simulink model "battery_cell_balancing_comparison"  (R2024b)
(part 3 of 4)

  EOL TWAICE Cell Model Pair 9 : batteryecm_lib/Battery (Table-Based)  Commented=on  SOC_vec=eol_soc  T_dependence=simscape.enum.tablebattery.temperature_dependence.yes  prm_dir=simscape.enum.tablebattery.prm_dir.noCurrentDirectionality  T_vec=temp_range degC  V0_mat=eol_ocv V  V0_vec=[3.5057, 3.566, 3.6337, 3.7127, 3.9259, 4.0777, 4.1928] V  V_range=[2.8,4.15] V  R0_mat=eol_ohmic_res mOhm  R0_vec=[.0085, .0085, .0087, .0082, .0083, .0085, .0085] Ohm  R0_dis_mat=[.0117, .0085, .009; .011, .0085, .009; .0114, .0087, .0092; .0107, .0082, .0088; .0107, .0083, .0091; .0113, .0085, .0089; .0116, .0085, .0089] Ohm  R0_dis_vec=[.0085, .0085, .0087, .0082, .0083, .0085, .0085] Ohm  R0_ch_mat=[.0117, .0085, .009; .011, .0085, .009; .0114, .0087, .0092; .0107, .0082, .0088; .0107, .0083, .0091; .0113, .0085, .0089; .0116, .0085, .0089] Ohm  R0_ch_vec=[.0085, .0085, .0087, .0082, .0083, .0085, .0085] Ohm  AH=eol_cell_cap A*hr  prm_leak=simscape.enum.tablebattery.prm_leak.disabled  Rleak_vec=[8000, 7000, 6000] Ohm  Rleak=7e3 Ohm  extrapolation_option=simscape.enum.extrapolation.linear  SOC_port=simscape.enum.tablebattery.enable.yes  prm_dyn=simscape.enum.tablebattery.prm_dyn.rc1  R1_mat=eol_first_pol_res mOhm  R1_vec=[.0029, .0024, .0026, .0016, .0023, .0018, .0017] Ohm  tau1_mat=eol_first_time_const s  tau1_vec=[36, 45, 105, 29, 77, 33, 39] s  R2_mat=[.0109, .0029, .0013; .0069, .0024, .0012; .0047, .0026, .0013; .0034, .0016, .001; .0033, .0023, .0014; .0033, .0018, .0011; .0028, .0017, .0011] Ohm  R2_vec=[.0029, .0024, .0026, .0016, .0023, .0018, .0017] Ohm  tau2_mat=[20, 36, 39; 31, 45, 39; 109, 105, 61; 36, 29, 26; 59, 77, 67; 40, 33, 29; 25, 39, 33] s  tau2_vec=[36, 45, 105, 29, 77, 33, 39] s  R3_mat=[.0109, .0029, .0013; .0069, .0024, .0012; .0047, .0026, .0013; .0034, .0016, .001; .0033, .0023, .0014; .0033, .0018, .0011; .0028, .0017, .0011] Ohm  R3_vec=[.0029, .0024, .0026, .0016, .0023, .0018, .0017] Ohm  tau3_mat=[20, 36, 39; 31, 45, 39; 109, 105, 61; 36, 29, 26; 59, 77, 67; 40, 33, 29; 25, 39, 33] s  tau3_vec=[36, 45, 105, 29, 77, 33, 39] s  R4_mat=[.0109, .0029, .0013; .0069, .0024, .0012; .0047, .0026, .0013; .0034, .0016, .001; .0033, .0023, .0014; .0033, .0018, .0011; .0028, .0017, .0011] Ohm  R4_vec=[.0029, .0024, .0026, .0016, .0023, .0018, .0017] Ohm  tau4_mat=[20, 36, 39; 31, 45, 39; 109, 105, 61; 36, 29, 26; 59, 77, 67; 40, 33, 29; 25, 39, 33] s  tau4_vec=[36, 45, 105, 29, 77, 33, 39] s  R5_mat=[.0109, .0029, .0013; .0069, .0024, .0012; .0047, .0026, .0013; .0034, .0016, .001; .0033, .0023, .0014; .0033, .0018, .0011; .0028, .0017, .0011] Ohm  R5_vec=[.0029, .0024, .0026, .0016, .0023, .0018, .0017] Ohm  tau5_mat=[20, 36, 39; 31, 45, 39; 109, 105, 61; 36, 29, 26; 59, 77, 67; 40, 33, 29; 25, 39, 33] s  tau5_vec=[36, 45, 105, 29, 77, 33, 39] s  prm_fade=simscape.enum.tablebattery.prm_fade.disabled  N0=100  dV0=0  dR0=0  dAH=0  dRleak=0  dR1=0  dR2=0  dR3=0  dR4=0  dR5=0  N0vec=[0, 100, 200, 300]  Tfadevec=[298.15, 323.15] K  dV0vec=[0, 0, 0, 0]  dR0vec=[0, 0, 0, 0]  dAHvec=[0, 0, 0, 0]  dRleakvec=[0, 0, 0, 0]  dR1vec=[0, 0, 0, 0]  dR2vec=[0, 0, 0, 0]  dR3vec=[0, 0, 0, 0]  dR4vec=[0, 0, 0, 0]  dR5vec=[0, 0, 0, 0]  dV0mat=[0, 0; 0, 0; 0, 0; 0, 0]  dR0mat=[0, 0; 0, 0; 0, 0; 0, 0]  dAHmat=[0, 0; 0, 0; 0, 0; 0, 0]  dRleakmat=[0, 0; 0, 0; 0, 0; 0, 0]  dR1mat=[0, 0; 0, 0; 0, 0; 0, 0]  dR2mat=[0, 0; 0, 0; 0, 0; 0, 0]  dR3mat=[0, 0; 0, 0; 0, 0; 0, 0]  dR4mat=[0, 0; 0, 0; 0, 0; 0, 0]  dR5mat=[0, 0; 0, 0; 0, 0; 0, 0]  prm_age_modeling=simscape.enum.tablebattery.prm_age_modeling.equation  storage_dt_age_vec=[0] d  storage_T_age_vec=[273] K  prm_age_OCV=simscape.enum.tablebattery.prm_age_OCV.OCV  OCV_age=0.9  SOC_age=0.6  prm_age_resistance=simscape.enum.tablebattery.prm_age.disabled  OCV_scaling_age_resistance=2.2134e6  OCV_offset_age_resistance=1.632e6  temp_exp_age_resistance=0.515833569 V  t_exp_age_resistance=0.75  T_age_vec_resistance=[273.15, 298.15, 323.15] K  dt_age_vec_resistance=[0, 90, 180, 270] d  dR0_age_vec=[0, 0, 0]  t_meas_dR0_age=100 d  dR0_age_mat=[0, 0, 0; 0, 0, 0; 0, 0, 0; 0, 0, 0]  prm_age_capacity=simscape.enum.tablebattery.prm_age.disabled  OCV_scaling_age_capacity=1.5097e07  OCV_offset_age_capacity=8.3625e06  temp_exp_age_capacity=0.6011 V  t_exp_age_capacity=0.75  T_age_vec_capacity=[273.15, 298.15, 323.15] K  dt_age_vec_capacity=[0, 90, 180, 270] d  dAH_age_vec=[0, 0, 0]  t_meas_dAH_age=100 d  dAH_age_mat=[0, 0, 0; 0, 0, 0; 0, 0, 0; 0, 0, 0]  thermal_port=simscape.enum.thermaleffects.omit  temperature=temp_init degC  thermal_mass=100 J/K  i_specify=off  i_priority=None  i=0 A  i_nominal_specify=off  i_nominal_value=1  i_nominal_unit=A  v_specify=on  v_priority=High  v=term_volt(9) V  v_nominal_specify=off  v_nominal_value=1  v_nominal_unit=V  stateOfCharge_specify=off  stateOfCharge_priority=High  stateOfCharge=1  stateOfCharge_nominal_specify=off  stateOfCharge_nominal_value=1  stateOfCharge_nominal_unit=1  num_cycles_specify=off  num_cycles_priority=High  num_cycles=0  num_cycles_nominal_specify=off  num_cycles_nominal_value=1  num_cycles_nominal_unit=1  cell_temperature_specify=off  cell_temperature_priority=High  cell_temperature=298.15 K  cell_temperature_nominal_specify=off  cell_temperature_nominal_value=1  cell_temperature_nominal_unit=K
      settings: InternalSimscapePortConfiguration="{\"Bottom\":[],\"Left\":[{\"id\":\"p\",\"label\":\"+\",\"type\":\"foundation.electrical.electrical\"},{\"id\":\"soc\",\"label\":\"SOC\",\"type\":\"output\"}],\"Right\":[{\"id\":\"n\",\"label\":\"-\",\"type\":\"foundation.electrical.electrical\"}],\"Top\":[]}"
  Electrical Reference : fl_lib/Electrical/Electrical Elements/Electrical Reference
  Electrical Reference1 : fl_lib/Electrical/Electrical Elements/Electrical Reference  Commented=on
  Electrical Reference2 : fl_lib/Electrical/Electrical Elements/Electrical Reference  Commented=on
  Electrical Reference4 : fl_lib/Electrical/Electrical Elements/Electrical Reference  Commented=on
  From : From  Commented=on  GotoTag=pack_voltage
  From104 : From  Commented=on  GotoTag=p2_volt
  From106 : From  Commented=on  GotoTag=p3_volt
  From107 : From  Commented=on  GotoTag=p4_volt
  From109 : From  Commented=on  GotoTag=p5_current
  From111 : From  Commented=on  GotoTag=p6_current
  From117 : From  Commented=on  GotoTag=p7_current
  From118 : From  Commented=on  GotoTag=p5_soc
  From120 : From  Commented=on  GotoTag=p11_cmd
  From122 : From  Commented=on  GotoTag=p6_soc
  From123 : From  Commented=on  GotoTag=p7_soc
  From124 : From  Commented=on  GotoTag=p8_soc
  From125 : From  Commented=on  GotoTag=p6_volt
  From126 : From  Commented=on  GotoTag=p7_volt
  From129 : From  Commented=on  GotoTag=p12_cmd
  From131 : From  Commented=on  GotoTag=p8_volt
  From133 : From  Commented=on  GotoTag=p9_current
  From135 : From  Commented=on  GotoTag=p10_current
  From136 : From  Commented=on  GotoTag=p11_current
  From142 : From  Commented=on  GotoTag=p12_current
  From144 : From  Commented=on  GotoTag=p5_cmd
  From146 : From  Commented=on  GotoTag=p9_soc
  From148 : From  Commented=on  GotoTag=p10_soc
  From149 : From  Commented=on  GotoTag=p11_soc
  From150 : From  Commented=on  GotoTag=p6_cmd
  From152 : From  Commented=on  GotoTag=p12_soc
  From154 : From  Commented=on  GotoTag=p9_volt
  From156 : From  Commented=on  GotoTag=p7_cmd
  From158 : From  Commented=on  GotoTag=p10_volt
  From159 : From  Commented=on  GotoTag=p11_volt
  From161 : From  Commented=on  GotoTag=p8_cmd
  From165 : From  Commented=on  GotoTag=p12_volt
  From166 : From  Commented=on  GotoTag=p5_cmd
  From167 : From  Commented=on  GotoTag=p6_cmd
  From168 : From  Commented=on  GotoTag=p7_cmd
  From169 : From  Commented=on  GotoTag=p8_cmd
  From170 : From  Commented=on  GotoTag=p4_current
  From171 : From  Commented=on  GotoTag=p3_soc
  From172 : From  Commented=on  GotoTag=p4_soc
  From173 : From  Commented=on  GotoTag=p1_volt
  From174 : From  Commented=on  GotoTag=p2_volt
  From175 : From  Commented=on  GotoTag=p3_volt
  From176 : From  Commented=on  GotoTag=p8_current
  From177 : From  Commented=on  GotoTag=p5_volt
  From178 : From  Commented=on  GotoTag=p4_volt
  From179 : From  Commented=on  GotoTag=p1_current
  From180 : From  Commented=on  GotoTag=p1_soc
  From{2..3,5,181,210} (5 alike) : From  Commented=on  GotoTag=pack_current
  From182 : From  Commented=on  GotoTag=p5_current
  From183 : From  Commented=on  GotoTag=p6_current
  From184 : From  Commented=on  GotoTag=p7_current
  From185 : From  Commented=on  GotoTag=p5_soc
  From186 : From  Commented=on  GotoTag=p11_cmd
  From187 : From  Commented=on  GotoTag=p6_soc
  From188 : From  Commented=on  GotoTag=p7_soc
  From189 : From  Commented=on  GotoTag=p8_soc
  From190 : From  Commented=on  GotoTag=p6_volt
  From191 : From  Commented=on  GotoTag=p7_volt
  From192 : From  Commented=on  GotoTag=p12_cmd
  From193 : From  Commented=on  GotoTag=p8_volt
  From194 : From  Commented=on  GotoTag=p9_current
  From195 : From  Commented=on  GotoTag=p10_current
  From196 : From  Commented=on  GotoTag=p11_current
  From197 : From  Commented=on  GotoTag=p12_current
  From198 : From  Commented=on  GotoTag=p9_soc
  From199 : From  Commented=on  GotoTag=p10_soc
  From200 : From  Commented=on  GotoTag=p11_soc
  From201 : From  Commented=on  GotoTag=p12_soc
  From202 : From  Commented=on  GotoTag=p9_volt
  From203 : From  Commented=on  GotoTag=p10_volt
  From204 : From  Commented=on  GotoTag=p11_volt
  From205 : From  Commented=on  GotoTag=p12_volt
  From206 : From  Commented=on  GotoTag=p8_current
  From207 : From  Commented=on  GotoTag=p5_volt
  From208 : From  Commented=on  GotoTag=p1_current
  From209 : From  Commented=on  GotoTag=p1_soc
  From211 : From  Commented=on  GotoTag=p3_current
  From212 : From  Commented=on  GotoTag=p2_soc
  From213 : From  Commented=on  GotoTag=p1_cmd
  From214 : From  Commented=on  GotoTag=p2_cmd
  From215 : From  Commented=on  GotoTag=p3_cmd
  From216 : From  Commented=on  GotoTag=p2_current
  From217 : From  Commented=on  GotoTag=p4_cmd
  From218 : From  Commented=on  GotoTag=p9_cmd
  From219 : From  Commented=on  GotoTag=p10_cmd
  From249 : From  Commented=on  GotoTag=p3_current
  From250 : From  Commented=on  GotoTag=p2_soc
  From251 : From  Commented=on  GotoTag=p1_cmd
  From252 : From  Commented=on  GotoTag=p2_cmd
  From253 : From  Commented=on  GotoTag=p3_cmd
  From254 : From  Commented=on  GotoTag=p2_current
  From255 : From  Commented=on  GotoTag=p4_cmd
  From256 : From  Commented=on  GotoTag=p9_cmd
  From257 : From  Commented=on  GotoTag=p10_cmd
  From258 : From  Commented=on  GotoTag=p4_current
  From259 : From  Commented=on  GotoTag=p3_soc
  From260 : From  Commented=on  GotoTag=p4_soc
  From261 : From  Commented=on  GotoTag=p1_volt
  From262 : From  Commented=on  GotoTag=p2_volt
  From263 : From  Commented=on  GotoTag=p3_volt
  From264 : From  Commented=on  GotoTag=p4_volt
  From265 : From  Commented=on  GotoTag=p5_current
  From266 : From  Commented=on  GotoTag=p6_current
  From267 : From  Commented=on  GotoTag=p7_current
  From268 : From  Commented=on  GotoTag=p5_soc
  From269 : From  Commented=on  GotoTag=p11_cmd
  From270 : From  Commented=on  GotoTag=p6_soc
  From271 : From  Commented=on  GotoTag=p7_soc
  From272 : From  Commented=on  GotoTag=p8_soc
  From273 : From  Commented=on  GotoTag=p6_volt
  From274 : From  Commented=on  GotoTag=p7_volt
  From275 : From  Commented=on  GotoTag=p12_cmd
  From276 : From  Commented=on  GotoTag=p8_volt
  From277 : From  Commented=on  GotoTag=p9_current
  From278 : From  Commented=on  GotoTag=p10_current
  From279 : From  Commented=on  GotoTag=p11_current
  From280 : From  Commented=on  GotoTag=p12_current
  From281 : From  Commented=on  GotoTag=p9_soc
  From282 : From  Commented=on  GotoTag=p10_soc
  From283 : From  Commented=on  GotoTag=p11_soc
  From284 : From  Commented=on  GotoTag=p12_soc
  From285 : From  Commented=on  GotoTag=p9_volt
  From286 : From  Commented=on  GotoTag=p10_volt
  From287 : From  Commented=on  GotoTag=p11_volt
  From288 : From  Commented=on  GotoTag=p12_volt
  From289 : From  Commented=on  GotoTag=p8_current
  From290 : From  Commented=on  GotoTag=p5_volt
  From291 : From  Commented=on  GotoTag=p1_current
  From292 : From  Commented=on  GotoTag=p1_soc
  From294 : From  Commented=on  GotoTag=p3_current
  From295 : From  Commented=on  GotoTag=p2_soc
  From296 : From  Commented=on  GotoTag=p1_cmd
  From297 : From  Commented=on  GotoTag=p2_cmd
  From298 : From  Commented=on  GotoTag=p3_cmd
  From299 : From  Commented=on  GotoTag=p2_current
  From300 : From  Commented=on  GotoTag=p4_cmd
  From301 : From  Commented=on  GotoTag=p9_cmd
  From302 : From  Commented=on  GotoTag=p10_cmd
  From4 : From  Commented=on  GotoTag=pack_voltage
  From87 : From  Commented=on  GotoTag=p5_cmd
  From93 : From  Commented=on  GotoTag=p6_cmd
  From94 : From  Commented=on  GotoTag=p7_cmd
  From95 : From  Commented=on  GotoTag=p8_cmd
  From96 : From  Commented=on  GotoTag=p4_current
  From97 : From  Commented=on  GotoTag=p3_soc
  From98 : From  Commented=on  GotoTag=p4_soc
  From99 : From  Commented=on  GotoTag=p1_volt
  Gain : Gain  Commented=on  Gain=2
  Gain1 : Gain  Commented=on  Gain=2
  Gain2 : Gain  Gain=2
  Goto1 : Goto  Commented=on  GotoTag=p1_cmd
  Goto10 : Goto  Commented=on  GotoTag=p10_cmd
  Goto103 : Goto  Commented=on  GotoTag=p9_soc
  Goto104 : Goto  Commented=on  GotoTag=p10_current
  Goto108 : Goto  Commented=on  GotoTag=p10_volt
  Goto109 : Goto  Commented=on  GotoTag=p11_soc
  Goto11 : Goto  Commented=on  GotoTag=p11_cmd
  Goto110 : Goto  Commented=on  GotoTag=p11_volt
  Goto112 : Goto  Commented=on  GotoTag=p11_current
  Goto115 : Goto  Commented=on  GotoTag=p12_soc
  Goto118 : Goto  Commented=on  GotoTag=p12_current
  Goto119 : Goto  Commented=on  GotoTag=p12_volt
  Goto12 : Goto  Commented=on  GotoTag=p12_cmd
  Goto122 : Goto  Commented=on  GotoTag=p9_volt
  Goto123 : Goto  Commented=on  GotoTag=p9_current
  Goto126 : Goto  Commented=on  GotoTag=p7_volt
  Goto127 : Goto  Commented=on  GotoTag=p10_soc
  Goto128 : Goto  Commented=on  GotoTag=p9_soc
  Goto129 : Goto  Commented=on  GotoTag=p10_current
  Goto13 : Goto  Commented=on  GotoTag=p1_cmd
  Goto130 : Goto  Commented=on  GotoTag=p10_volt
  Goto131 : Goto  Commented=on  GotoTag=p11_soc
  Goto132 : Goto  Commented=on  GotoTag=p11_volt
  Goto133 : Goto  Commented=on  GotoTag=p11_current
  Goto134 : Goto  Commented=on  GotoTag=p12_soc
  Goto135 : Goto  Commented=on  GotoTag=p12_current
  Goto136 : Goto  Commented=on  GotoTag=p12_volt
  Goto137 : Goto  Commented=on  GotoTag=p9_volt
  Goto138 : Goto  Commented=on  GotoTag=p9_current
  Goto139 : Goto  Commented=on  GotoTag=pack_current
  Goto14 : Goto  Commented=on  GotoTag=p2_cmd
  Goto140 : Goto  Commented=on  GotoTag=p1_current
  Goto141 : Goto  Commented=on  GotoTag=p2_soc
  Goto142 : Goto  Commented=on  GotoTag=p1_soc
  Goto145 : Goto  Commented=on  GotoTag=p2_current
  Goto146 : Goto  Commented=on  GotoTag=p2_volt
  Goto147 : Goto  Commented=on  GotoTag=p6_current
  Goto148 : Goto  Commented=on  GotoTag=p3_soc
  Goto15 : Goto  Commented=on  GotoTag=p3_cmd
  Goto151 : Goto  Commented=on  GotoTag=p3_volt
  Goto153 : Goto  Commented=on  GotoTag=pack_voltage
  Goto154 : Goto  Commented=on  GotoTag=p3_current
  Goto155 : Goto  Commented=on  GotoTag=p4_soc
  Goto157 : Goto  Commented=on  GotoTag=p4_current
  Goto158 : Goto  Commented=on  GotoTag=p4_volt
  Goto159 : Goto  Commented=on  GotoTag=p6_volt
  Goto16 : Goto  Commented=on  GotoTag=p4_cmd
  Goto162 : Goto  Commented=on  GotoTag=p5_current
  Goto163 : Goto  Commented=on  GotoTag=p5_soc
  Goto165 : Goto  Commented=on  GotoTag=p6_soc
  Goto166 : Goto  Commented=on  GotoTag=p8_current
  Goto169 : Goto  Commented=on  GotoTag=p8_volt
  Goto17 : Goto  Commented=on  GotoTag=p5_cmd
  Goto171 : Goto  Commented=on  GotoTag=p7_current
  Goto172 : Goto  Commented=on  GotoTag=p7_soc
  Goto173 : Goto  Commented=on  GotoTag=p8_soc
  Goto174 : Goto  Commented=on  GotoTag=p1_volt
  Goto175 : Goto  Commented=on  GotoTag=p5_volt
  Goto18 : Goto  Commented=on  GotoTag=p6_cmd
  Goto189 : Goto  Commented=on  GotoTag=pack_current
  Goto19 : Goto  Commented=on  GotoTag=p7_cmd
  Goto190 : Goto  Commented=on  GotoTag=p1_current
  Goto191 : Goto  Commented=on  GotoTag=p2_soc
  Goto192 : Goto  Commented=on  GotoTag=p1_soc
  Goto195 : Goto  Commented=on  GotoTag=p2_current
  Goto196 : Goto  Commented=on  GotoTag=p2_volt
  Goto197 : Goto  Commented=on  GotoTag=p6_current
  Goto198 : Goto  Commented=on  GotoTag=p3_soc
  Goto2 : Goto  Commented=on  GotoTag=p2_cmd
  Goto20 : Goto  Commented=on  GotoTag=p8_cmd
  Goto201 : Goto  Commented=on  GotoTag=p3_volt
  Goto203 : Goto  Commented=on  GotoTag=pack_voltage
  Goto204 : Goto  Commented=on  GotoTag=p3_current
  Goto205 : Goto  Commented=on  GotoTag=p4_soc
  Goto207 : Goto  Commented=on  GotoTag=p4_current
  Goto208 : Goto  Commented=on  GotoTag=p4_volt
  Goto209 : Goto  Commented=on  GotoTag=p6_volt
  Goto21 : Goto  Commented=on  GotoTag=p9_cmd
  Goto212 : Goto  Commented=on  GotoTag=p5_current
  Goto213 : Goto  Commented=on  GotoTag=p5_soc
  Goto215 : Goto  Commented=on  GotoTag=p6_soc
  Goto216 : Goto  Commented=on  GotoTag=p8_current
  Goto219 : Goto  Commented=on  GotoTag=p8_volt
  Goto22 : Goto  Commented=on  GotoTag=p10_cmd
  Goto221 : Goto  Commented=on  GotoTag=p7_current
  Goto222 : Goto  Commented=on  GotoTag=p7_soc
  Goto223 : Goto  Commented=on  GotoTag=p8_soc
  Goto224 : Goto  Commented=on  GotoTag=p1_volt
  Goto225 : Goto  Commented=on  GotoTag=p5_volt
  Goto226 : Goto  Commented=on  GotoTag=p7_volt
  Goto227 : Goto  Commented=on  GotoTag=p10_soc
  Goto228 : Goto  Commented=on  GotoTag=p9_soc
  Goto229 : Goto  Commented=on  GotoTag=p10_current
  Goto23 : Goto  Commented=on  GotoTag=p11_cmd
  Goto230 : Goto  Commented=on  GotoTag=p10_volt
  Goto231 : Goto  Commented=on  GotoTag=p11_soc
  Goto232 : Goto  Commented=on  GotoTag=p11_volt
  Goto233 : Goto  Commented=on  GotoTag=p11_current
  Goto234 : Goto  Commented=on  GotoTag=p12_soc
  Goto235 : Goto  Commented=on  GotoTag=p12_current
  Goto236 : Goto  Commented=on  GotoTag=p12_volt
  Goto237 : Goto  Commented=on  GotoTag=p9_volt
  Goto238 : Goto  Commented=on  GotoTag=p9_current
  Goto239 : Goto  Commented=on  GotoTag=pack_current
  Goto24 : Goto  Commented=on  GotoTag=p12_cmd
  Goto240 : Goto  Commented=on  GotoTag=p1_current
  Goto241 : Goto  Commented=on  GotoTag=p2_soc
  Goto242 : Goto  Commented=on  GotoTag=p1_soc
  Goto243 : Goto  Commented=on  GotoTag=p1_cmd
  Goto244 : Goto  Commented=on  GotoTag=p2_cmd
  Goto245 : Goto  Commented=on  GotoTag=p2_current
  Goto246 : Goto  Commented=on  GotoTag=p2_volt
  Goto247 : Goto  Commented=on  GotoTag=p6_current
  Goto248 : Goto  Commented=on  GotoTag=p3_soc
  Goto249 : Goto  Commented=on  GotoTag=p3_cmd
  Goto250 : Goto  Commented=on  GotoTag=p4_cmd
  Goto251 : Goto  Commented=on  GotoTag=p3_volt
  Goto252 : Goto  Commented=on  GotoTag=p5_cmd
  Goto253 : Goto  Commented=on  GotoTag=pack_voltage
  Goto254 : Goto  Commented=on  GotoTag=p3_current
  Goto255 : Goto  Commented=on  GotoTag=p4_soc
  Goto256 : Goto  Commented=on  GotoTag=p6_cmd
  Goto257 : Goto  Commented=on  GotoTag=p4_current
  Goto258 : Goto  Commented=on  GotoTag=p4_volt
  Goto259 : Goto  Commented=on  GotoTag=p6_volt
  Goto260 : Goto  Commented=on  GotoTag=p7_cmd
  Goto261 : Goto  Commented=on  GotoTag=p8_cmd
  Goto262 : Goto  Commented=on  GotoTag=p5_current
  Goto263 : Goto  Commented=on  GotoTag=p5_soc
  Goto264 : Goto  Commented=on  GotoTag=p9_cmd
  Goto265 : Goto  Commented=on  GotoTag=p6_soc
  Goto266 : Goto  Commented=on  GotoTag=p8_current
  Goto267 : Goto  Commented=on  GotoTag=p10_cmd
  Goto268 : Goto  Commented=on  GotoTag=p11_cmd
  Goto269 : Goto  Commented=on  GotoTag=p8_volt
  Goto270 : Goto  Commented=on  GotoTag=p12_cmd
  Goto271 : Goto  Commented=on  GotoTag=p7_current
  Goto272 : Goto  Commented=on  GotoTag=p7_soc
  Goto273 : Goto  Commented=on  GotoTag=p8_soc
  Goto274 : Goto  Commented=on  GotoTag=p1_volt
  Goto275 : Goto  Commented=on  GotoTag=p5_volt
  Goto3 : Goto  Commented=on  GotoTag=p3_cmd
  Goto4 : Goto  Commented=on  GotoTag=p4_cmd
  Goto5 : Goto  Commented=on  GotoTag=p5_cmd
  Goto6 : Goto  Commented=on  GotoTag=p6_cmd
  Goto7 : Goto  Commented=on  GotoTag=p7_cmd
  Goto8 : Goto  Commented=on  GotoTag=p8_cmd
  Goto9 : Goto  Commented=on  GotoTag=p9_cmd
  Goto96 : Goto  Commented=on  GotoTag=p7_volt
  Goto98 : Goto  Commented=on  GotoTag=p10_soc
  MT42 Capacitance1 : fl_lib/Electrical/Electrical Elements/Capacitor  c=11 mF  r=1e-6 Ohm  g=0 1/Ohm  i_specify=off  i_priority=None  i=0 A  i_nominal_specify=off  i_nominal_value=1  i_nominal_unit=A  v_specify=off  v_priority=None  v=0 V  v_nominal_specify=off  v_nominal_value=1  v_nominal_unit=V  vc_specify=off  vc_priority=High  vc=0 V  vc_nominal_specify=off  vc_nominal_value=1  vc_nominal_unit=V
  MT42 Capacitance2 : fl_lib/Electrical/Electrical Elements/Capacitor  Commented=on  c=11 mF  r=1e-6 Ohm  g=0 1/Ohm  i_specify=off  i_priority=None  i=0 A  i_nominal_specify=off  i_nominal_value=1  i_nominal_unit=A  v_specify=off  v_priority=None  v=0 V  v_nominal_specify=off  v_nominal_value=1  v_nominal_unit=V  vc_specify=off  vc_priority=High  vc=0 V  vc_nominal_specify=off  vc_nominal_value=1  vc_nominal_unit=V
  MT42 Capacitance3 : fl_lib/Electrical/Electrical Elements/Capacitor  Commented=on  c=11 mF  r=1e-6 Ohm  g=0 1/Ohm  i_specify=off  i_priority=None  i=0 A  i_nominal_specify=off  i_nominal_value=1  i_nominal_unit=A  v_specify=off  v_priority=None  v=0 V  v_nominal_specify=off  v_nominal_value=1  v_nominal_unit=V  vc_specify=off  vc_priority=High  vc=0 V  vc_nominal_specify=off  vc_nominal_value=1  vc_nominal_unit=V
  MT42 Capacitance4 : fl_lib/Electrical/Electrical Elements/Capacitor  Commented=on  c=11 mF  r=1e-6 Ohm  g=0 1/Ohm  i_specify=off  i_priority=None  i=0 A  i_nominal_specify=off  i_nominal_value=1  i_nominal_unit=A  v_specify=off  v_priority=None  v=0 V  v_nominal_specify=off  v_nominal_value=1  v_nominal_unit=V  vc_specify=off  vc_priority=High  vc=0 V  vc_nominal_specify=off  vc_nominal_value=1  vc_nominal_unit=V
  PS-Simulink Converter{63..64,67,69,71,73..75,77..78,80..81,83..84,86,89,91..92,94..97,100..101,104..105,107..110,112,114,116..117,120,123} (36 alike) : nesl_utility/PS-Simulink Converter  PhysicalDomain=network_engine_domain  SubClassName=ps_output  LeftPortType=input  RightPortType=output  PseudoPeriodic=off  Frequencies=[]  VectorFormat=inherit  Unit=inherit  AffineConversion=off
  PS-Simulink Converter102 : nesl_utility/PS-Simulink Converter  Commented=on  PhysicalDomain=network_engine_domain  SubClassName=ps_output  LeftPortType=input  RightPortType=output  PseudoPeriodic=off  Frequencies=[]  VectorFormat=inherit  Unit=V  AffineConversion=on
  PS-Simulink Converter{65..66,68,70,72,76,79,82,85,87..88,90,93,99,103,106,111,113,115,118..119,121,124..136,138,140..161,186..212,214,216..237} (108 alike) : nesl_utility/PS-Simulink Converter  Commented=on  PhysicalDomain=network_engine_domain  SubClassName=ps_output  LeftPortType=input  RightPortType=output  PseudoPeriodic=off  Frequencies=[]  VectorFormat=inherit  Unit=inherit  AffineConversion=off
  PS-Simulink Converter122 : nesl_utility/PS-Simulink Converter  PhysicalDomain=network_engine_domain  SubClassName=ps_output  LeftPortType=input  RightPortType=output  PseudoPeriodic=off  Frequencies=[]  VectorFormat=inherit  Unit=A  AffineConversion=on
  PS-Simulink Converter137 : nesl_utility/PS-Simulink Converter  Commented=on  PhysicalDomain=network_engine_domain  SubClassName=ps_output  LeftPortType=input  RightPortType=output  PseudoPeriodic=off  Frequencies=[]  VectorFormat=inherit  Unit=A  AffineConversion=on
  PS-Simulink Converter139 : nesl_utility/PS-Simulink Converter  Commented=on  PhysicalDomain=network_engine_domain  SubClassName=ps_output  LeftPortType=input  RightPortType=output  PseudoPeriodic=off  Frequencies=[]  VectorFormat=inherit  Unit=V  AffineConversion=on
  PS-Simulink Converter213 : nesl_utility/PS-Simulink Converter  Commented=on  PhysicalDomain=network_engine_domain  SubClassName=ps_output  LeftPortType=input  RightPortType=output  PseudoPeriodic=off  Frequencies=[]  VectorFormat=inherit  Unit=A  AffineConversion=on
  PS-Simulink Converter215 : nesl_utility/PS-Simulink Converter  Commented=on  PhysicalDomain=network_engine_domain  SubClassName=ps_output  LeftPortType=input  RightPortType=output  PseudoPeriodic=off  Frequencies=[]  VectorFormat=inherit  Unit=V  AffineConversion=on
  PS-Simulink Converter62 : nesl_utility/PS-Simulink Converter  PhysicalDomain=network_engine_domain  SubClassName=ps_output  LeftPortType=input  RightPortType=output  PseudoPeriodic=off  Frequencies=[]  VectorFormat=inherit  Unit=V  AffineConversion=on
  PS-Simulink Converter98 : nesl_utility/PS-Simulink Converter  Commented=on  PhysicalDomain=network_engine_domain  SubClassName=ps_output  LeftPortType=input  RightPortType=output  PseudoPeriodic=off  Frequencies=[]  VectorFormat=inherit  Unit=A  AffineConversion=on
  Pulse Generator1 : DiscretePulseGenerator  Commented=on  PulseType=Time based  Period=60  PulseWidth=5
  Pulse Generator2 : DiscretePulseGenerator  PulseType=Time based  Period=60  PulseWidth=5
  Pulse Generator3 : DiscretePulseGenerator  Commented=on  PulseType=Time based  Period=60  PulseWidth=5
  Pulse Generator5 : DiscretePulseGenerator  Commented=on  PulseType=Time based  Period=60  PulseWidth=5
  Repeating Sequence : simulink/Sources/Repeating Sequence  Commented=on  rep_seq_t=udds_val_time  rep_seq_y=udds_val_current_profile
  Repeating Sequence1 : simulink/Sources/Repeating Sequence  Commented=on  rep_seq_t=udds_val_time  rep_seq_y=udds_val_current_profile
  Repeating Sequence2 : simulink/Sources/Repeating Sequence  rep_seq_t=udds_val_time  rep_seq_y=udds_val_current_profile
  Resistor{13..19,21..25} (12 alike) : fl_lib/Electrical/Electrical Elements/Resistor  R=5 Ohm  i_specify=off  i_priority=None  i=0 A  i_nominal_specify=off  i_nominal_value=1  i_nominal_unit=A  v_specify=off  v_priority=None  v=0 V  v_nominal_specify=off  v_nominal_value=1  v_nominal_unit=V
  Resistor20 : fl_lib/Electrical/Electrical Elements/Resistor  R=100 Ohm  i_specify=off  i_priority=None  i=0 A  i_nominal_specify=off  i_nominal_value=1  i_nominal_unit=A  v_specify=off  v_priority=None  v=0 V  v_nominal_specify=off  v_nominal_value=1  v_nominal_unit=V
  Resistor{26..32,34..45,47..58,60..64} (36 alike) : fl_lib/Electrical/Electrical Elements/Resistor  Commented=on  R=5 Ohm  i_specify=off  i_priority=None  i=0 A  i_nominal_specify=off  i_nominal_value=1  i_nominal_unit=A  v_specify=off  v_priority=None  v=0 V  v_nominal_specify=off  v_nominal_value=1  v_nominal_unit=V
  Resistor33 : fl_lib/Electrical/Electrical Elements/Resistor  Commented=on  R=100 Ohm  i_specify=off  i_priority=None  i=0 A  i_nominal_specify=off  i_nominal_value=1  i_nominal_unit=A  v_specify=off  v_priority=None  v=0 V  v_nominal_specify=off  v_nominal_value=1  v_nominal_unit=V
  Resistor46 : fl_lib/Electrical/Electrical Elements/Resistor  Commented=on  R=100 Ohm  i_specify=off  i_priority=None  i=0 A  i_nominal_specify=off  i_nominal_value=1  i_nominal_unit=A  v_specify=off  v_priority=None  v=0 V  v_nominal_specify=off  v_nominal_value=1  v_nominal_unit=V
  Resistor59 : fl_lib/Electrical/Electrical Elements/Resistor  Commented=on  R=100 Ohm  i_specify=off  i_priority=None  i=0 A  i_nominal_specify=off  i_nominal_value=1  i_nominal_unit=A  v_specify=off  v_priority=None  v=0 V  v_nominal_specify=off  v_nominal_value=1  v_nominal_unit=V
  SPST Switch{14..27} (14 alike) : ee_lib/Switches & Breakers/SPST Switch  R_closed=0.01 Ohm  G_open=1e-6 S  Threshold=0.5 V  Width=0 V  model_dynamics=0  t_on=1e-3 s  t_off=1e-3 s  initial_vT=0 V
      settings: InternalSimscapePortConfiguration="{\"Bottom\":[],\"Left\":[{\"id\":\"vT\",\"label\":\"vT\",\"type\":\"input\"},{\"id\":\"p\",\"label\":\"\",\"type\":\"foundation.electrical.electrical\"}],\"Right\":[{\"id\":\"n\",\"label\":\"\",\"type\":\"foundation.electrical.electrical\"}],\"Top\":[]}"
  SPST Switch{28..69} (42 alike) : ee_lib/Switches & Breakers/SPST Switch  Commented=on  R_closed=0.01 Ohm  G_open=1e-6 S  Threshold=0.5 V  Width=0 V  model_dynamics=0  t_on=1e-3 s  t_off=1e-3 s  initial_vT=0 V
      settings: InternalSimscapePortConfiguration="{\"Bottom\":[],\"Left\":[{\"id\":\"vT\",\"label\":\"vT\",\"type\":\"input\"},{\"id\":\"p\",\"label\":\"\",\"type\":\"foundation.electrical.electrical\"}],\"Right\":[{\"id\":\"n\",\"label\":\"\",\"type\":\"foundation.electrical.electrical\"}],\"Top\":[]}"
  Scope : Scope  Commented=on  NumInputPorts=2
  Scope1 : Scope  NumInputPorts=4
  Scope2 : Scope  Commented=on  NumInputPorts=4
  Scope3 : Scope  Commented=on  NumInputPorts=4
  Scope4 : Scope  Commented=on  NumInputPorts=4
  Scope5 : Scope  Commented=on  NumInputPorts=2
  Scope6 : Scope  NumInputPorts=2
  Simulink-PS Converter{15..29} (15 alike) : nesl_utility/Simulink-PS Converter  PhysicalDomain=network_engine_domain  SubClassName=ps_input  LeftPortType=input  RightPortType=output  PseudoPeriodic=off  Frequencies=[]  NoiseDistribution=none  NoiseParameters=[]  Unit=1  AffineConversion=off  FilteringAndDerivatives=provide  SimscapeFilterOrder=1  InputFilterTimeConstant=0.001  UdotUserProvided=0
  Simulink-PS Converter{30..74} (45 alike) : nesl_utility/Simulink-PS Converter  Commented=on  PhysicalDomain=network_engine_domain  SubClassName=ps_input  LeftPortType=input  RightPortType=output  PseudoPeriodic=off  Frequencies=[]  NoiseDistribution=none  NoiseParameters=[]  Unit=1  AffineConversion=off  FilteringAndDerivatives=provide  SimscapeFilterOrder=1  InputFilterTimeConstant=0.001  UdotUserProvided=0
  Solver Configuration : nesl_utility/Solver Configuration  PhysicalDomain=network_engine_domain  SubClassName=solver  LeftPortType=input  RightPortType=generic  Tones=[]  Harmonics=[]  SimulateNoise=off  Profile=off  UseLocalSampling=off  EnableSwitchedLinearOptims=on  FrequencyDomain=off  UseCCode=off  RelTol=0.001  AbsTol=0.001  MinStep=1e-09  ToWorkspace=off  RevertToSquareIcSolve=off  NumHomotopyIterations=100  PhasorMode=off  PhasorModeNumHarmonics=1  ConsistencySolver=NEWTON_XTOL_AFTER_FTOL  IndexReductionMethod=DerivativeReplacement  DoDC=off  ResidualTolerance=1e-09  ConsistencyTolSource=GLOBAL  ConsistencyAbsTol=0.001  ConsistencyRelTol=0.001  ConsistencyTolFactor=0.001  UseLocalSolver=off  LocalSolverChoice=NE_BACKWARD_EULER_ADVANCER  ResolveIndetEquations=on  FunctionEvalNumThread=1  LocalSolverSampleTime=0.001  DoFixedCost=off  MaxNonlinIter=3  MaxModeIter=2  ComputeImpulses=off  ImpulseIterations=2  LinearAlgebra=auto  LinearAlgebraNumThread=0  EquationFormulation=NE_TIME_EF  DelaysMemoryBudget=1024  AutomaticFiltering=on  FilteringTimeConstant=0.001  PartitionStorageMethod=AS_NEEDED  PartitionMemoryBudget=1024  PartitionMethod=ROBUST  MultibodyUseLocalSolver=off  MultibodyLocalSolverChoice=ODE1  MultibodyLocalSolverSampleTime=0.001
  Solver Configuration2 : nesl_utility/Solver Configuration  Commented=on  PhysicalDomain=network_engine_domain  SubClassName=solver  LeftPortType=input  RightPortType=generic  Tones=[]  Harmonics=[]  SimulateNoise=off  Profile=off  UseLocalSampling=off  EnableSwitchedLinearOptims=on  FrequencyDomain=off  UseCCode=off  RelTol=0.001  AbsTol=0.001  MinStep=1e-09  ToWorkspace=off  RevertToSquareIcSolve=off  NumHomotopyIterations=100  PhasorMode=off  PhasorModeNumHarmonics=1  ConsistencySolver=NEWTON_XTOL_AFTER_FTOL  IndexReductionMethod=DerivativeReplacement  DoDC=off  ResidualTolerance=1e-09  ConsistencyTolSource=GLOBAL  ConsistencyAbsTol=0.001  ConsistencyRelTol=0.001  ConsistencyTolFactor=0.001  UseLocalSolver=off  LocalSolverChoice=NE_BACKWARD_EULER_ADVANCER  ResolveIndetEquations=on  FunctionEvalNumThread=1  LocalSolverSampleTime=0.001  DoFixedCost=off  MaxNonlinIter=3  MaxModeIter=2  ComputeImpulses=off  ImpulseIterations=2  LinearAlgebra=auto  LinearAlgebraNumThread=0  EquationFormulation=NE_TIME_EF  DelaysMemoryBudget=1024  AutomaticFiltering=on  FilteringTimeConstant=0.001  PartitionStorageMethod=AS_NEEDED  PartitionMemoryBudget=1024  PartitionMethod=ROBUST  MultibodyUseLocalSolver=off  MultibodyLocalSolverChoice=ODE1  MultibodyLocalSolverSampleTime=0.001
  Solver Configuration3 : nesl_utility/Solver Configuration  Commented=on  PhysicalDomain=network_engine_domain  SubClassName=solver  LeftPortType=input  RightPortType=generic  Tones=[]  Harmonics=[]  SimulateNoise=off  Profile=off  UseLocalSampling=off  EnableSwitchedLinearOptims=on  FrequencyDomain=off  UseCCode=off  RelTol=0.001  AbsTol=0.001  MinStep=1e-09  ToWorkspace=off  RevertToSquareIcSolve=off  NumHomotopyIterations=100  PhasorMode=off  PhasorModeNumHarmonics=1  ConsistencySolver=NEWTON_XTOL_AFTER_FTOL  IndexReductionMethod=DerivativeReplacement  DoDC=off  ResidualTolerance=1e-09  ConsistencyTolSource=GLOBAL  ConsistencyAbsTol=0.001  ConsistencyRelTol=0.001  ConsistencyTolFactor=0.001  UseLocalSolver=off  LocalSolverChoice=NE_BACKWARD_EULER_ADVANCER  ResolveIndetEquations=on  FunctionEvalNumThread=1  LocalSolverSampleTime=0.001  DoFixedCost=off  MaxNonlinIter=3  MaxModeIter=2  ComputeImpulses=off  ImpulseIterations=2  LinearAlgebra=auto  LinearAlgebraNumThread=0  EquationFormulation=NE_TIME_EF  DelaysMemoryBudget=1024  AutomaticFiltering=on  FilteringTimeConstant=0.001  PartitionStorageMethod=AS_NEEDED  PartitionMemoryBudget=1024  PartitionMethod=ROBUST  MultibodyUseLocalSolver=off  MultibodyLocalSolverChoice=ODE1  MultibodyLocalSolverSampleTime=0.001
  Solver Configuration4 : nesl_utility/Solver Configuration  Commented=on  PhysicalDomain=network_engine_domain  SubClassName=solver  LeftPortType=input  RightPortType=generic  Tones=[]  Harmonics=[]  SimulateNoise=off  Profile=off  UseLocalSampling=off  EnableSwitchedLinearOptims=on  FrequencyDomain=off  UseCCode=off  RelTol=0.001  AbsTol=0.001  MinStep=1e-09  ToWorkspace=off  RevertToSquareIcSolve=off  NumHomotopyIterations=100  PhasorMode=off  PhasorModeNumHarmonics=1  ConsistencySolver=NEWTON_XTOL_AFTER_FTOL  IndexReductionMethod=DerivativeReplacement  DoDC=off  ResidualTolerance=1e-09  ConsistencyTolSource=GLOBAL  ConsistencyAbsTol=0.001  ConsistencyRelTol=0.001  ConsistencyTolFactor=0.001  UseLocalSolver=off  LocalSolverChoice=NE_BACKWARD_EULER_ADVANCER  ResolveIndetEquations=on  FunctionEvalNumThread=1  LocalSolverSampleTime=0.001  DoFixedCost=off  MaxNonlinIter=3  MaxModeIter=2  ComputeImpulses=off  ImpulseIterations=2  LinearAlgebra=auto  LinearAlgebraNumThread=0  EquationFormulation=NE_TIME_EF  DelaysMemoryBudget=1024  AutomaticFiltering=on  FilteringTimeConstant=0.001  PartitionStorageMethod=AS_NEEDED  PartitionMemoryBudget=1024  PartitionMethod=ROBUST  MultibodyUseLocalSolver=off  MultibodyLocalSolverChoice=ODE1  MultibodyLocalSolverSampleTime=0.001
  Step1 : Step  Commented=on  Time=10
  Step10 : Step  Commented=on  Time=10
  Step11 : Step  Time=10
  Step2 : Step  Time=5
  Step3 : Step  Time=6  Before=1  After=0
  Step4 : Step  Commented=on  Time=5
  Step5 : Step  Commented=on  Time=6  Before=1  After=0
  Step6 : Step  Commented=on  Time=5
  Step7 : Step  Commented=on  Time=6  Before=1  After=0
  Step8 : Step  Commented=on  Time=5
  Step9 : Step  Commented=on  Time=6  Before=1  After=0
  Switch : Switch  Commented=on  Criteria=u2 > Threshold  SaturateOnIntegerOverflow=off  InputSameDT=off
  Switch1 : Switch  Commented=on  Criteria=u2 > Threshold  SaturateOnIntegerOverflow=off  InputSameDT=off
  Switch2 : Switch  Criteria=u2 > Threshold  SaturateOnIntegerOverflow=off  InputSameDT=off
  To File : ToFile  Commented=on  Filename=cell_voltages.mat  MatrixName=cell_voltages  SampleTime=60
  To File1 : ToFile  Commented=on  Filename=cell_balance_cmd.mat  MatrixName=cell_balance_cmd  SampleTime=60
  To File2 : ToFile  Commented=on  Filename=cell_voltages.mat  MatrixName=cell_voltages  SampleTime=60
  To File3 : ToFile  Commented=on  Filename=cell_balance_cmd.mat  MatrixName=cell_balance_cmd  SampleTime=60
  To File4 : ToFile  Filename=cell_voltages.mat  MatrixName=cell_voltages  SampleTime=60
  To File5 : ToFile  Filename=cell_balance_cmd.mat  MatrixName=cell_balance_cmd  SampleTime=60
  Voltage Sensor{13..18,20..25,39} (13 alike) : fl_lib/Electrical/Electrical Sensors/Voltage Sensor
  Voltage Sensor{19,26..38,40..64} (39 alike) : fl_lib/Electrical/Electrical Sensors/Voltage Sensor  Commented=on
  balancing1 : MATLAB Function  TreatAsAtomicUnit=on
  balancing2 : MATLAB Function  Commented=on  TreatAsAtomicUnit=on
  balancing3 : MATLAB Function  Commented=on  TreatAsAtomicUnit=on
  balancing5 : MATLAB Function  Commented=on  TreatAsAtomicUnit=on
  wires:
  [p12_current] -> Bus Creator12/12  "p12_current"
  PS-Simulink Converter91/1 -> [p8_soc]
  PS-Simulink Converter94/1 -> [p8_volt]
  PS-Simulink Converter92/1 -> [p7_soc]
  [p8_cmd] -> Data Type Conversion7/1
  PS-Simulink Converter77/1 -> [p6_soc]
  [p6_cmd] -> Data Type Conversion5/1
  PS-Simulink Converter116/1 -> [p9_volt]
  PS-Simulink Converter105/1 -> [p11_volt]
  PS-Simulink Converter120/1 -> [p9_current]
  PS-Simulink Converter117/1 -> [p10_volt]
  PS-Simulink Converter104/1 -> [p11_soc]
  [p11_cmd] -> Data Type Conversion10/1
  PS-Simulink Converter114/1 -> [p12_volt]
  [p10_cmd] -> Data Type Conversion9/1
  [p3_soc] -> Bus Creator10/3  "p3_soc"
  PS-Simulink Converter110/1 -> [p12_current]
  [p9_soc] -> Bus Creator10/9  "p9_soc"
  [p10_soc] -> Bus Creator10/10  "p10_soc"
  [p8_soc] -> Bus Creator10/8  "p8_soc"
  PS-Simulink Converter95/1 -> [p7_volt]
  [p5_soc] -> Bus Creator10/5  "p5_soc"
  [p7_current] -> Bus Creator12/7  "p7_current"
  [p12_volt] -> Bus Creator11/12  "p12_volt"
  PS-Simulink Converter108/1 -> [p11_current]
  [p3_current] -> Bus Creator12/3  "p3_current"
  [p9_volt] -> Bus Creator11/9  "p9_volt"
  [p11_volt] -> Bus Creator11/11  "p11_volt"
  [p6_volt] -> Bus Creator11/6  "p6_volt"
  [p4_current] -> Bus Creator12/4  "p4_current"
  PS-Simulink Converter101/1 -> [p10_current]
  PS-Simulink Converter80/1 -> [p4_volt]
  PS-Simulink Converter75/1 -> [p4_current]
  PS-Simulink Converter78/1 -> [p4_soc]
  PS-Simulink Converter89/1 -> [p8_current]
  [p1_volt] -> Bus Creator11/1  "p1_volt"
  [p2_volt] -> Bus Creator11/2  "p2_volt"
  [p3_volt] -> Bus Creator11/3  "p3_volt"
  PS-Simulink Converter86/1 -> [p5_current]
  [p4_volt] -> Bus Creator11/4  "p4_volt"
  [p2_soc] -> Bus Creator10/2  "p2_soc"
  PS-Simulink Converter84/1 -> [p5_volt]
  [p6_current] -> Bus Creator12/6  "p6_current"
  PS-Simulink Converter100/1 -> [p9_soc]
  PS-Simulink Converter97/1 -> [p7_current]
  [p7_cmd] -> Data Type Conversion6/1
  PS-Simulink Converter83/1 -> [p6_volt]
  PS-Simulink Converter107/1 -> [p2_volt]
  [p2_current] -> Bus Creator12/2  "p2_current"
  [p10_volt] -> Bus Creator11/10  "p10_volt"
  PS-Simulink Converter81/1 -> [p5_soc]
  PS-Simulink Converter73/1 -> [p3_current]
  [p5_current] -> Bus Creator12/5  "p5_current"
  PS-Simulink Converter69/1 -> [p3_soc]
  PS-Simulink Converter71/1 -> [p3_volt]
  [p11_soc] -> Bus Creator10/11  "p11_soc"
  [p9_current] -> Bus Creator12/9  "p9_current"
  PS-Simulink Converter112/1 -> [p12_soc]
  [p6_soc] -> Bus Creator10/6  "p6_soc"
  [p5_cmd] -> Data Type Conversion4/1
  [p11_current] -> Bus Creator12/11  "p11_current"
  [p8_current] -> Bus Creator12/8  "p8_current"
  PS-Simulink Converter67/1 -> [p6_current]
  PS-Simulink Converter74/1 -> [p2_soc]
  PS-Simulink Converter64/1 -> [p2_current]
  [p5_volt] -> Bus Creator11/5  "p5_volt"
  [p7_volt] -> Bus Creator11/7  "p7_volt"
  [p4_soc] -> Bus Creator10/4  "p4_soc"
  [p8_volt] -> Bus Creator11/8  "p8_volt"
  PS-Simulink Converter96/1 -> [p1_volt]
  [p9_cmd] -> Data Type Conversion8/1
  PS-Simulink Converter63/1 -> [p1_soc]
  [p1_current] -> Bus Creator12/1  "p1_current"
  PS-Simulink Converter122/1 -> [pack_current]
  [p12_soc] -> Bus Creator10/12  "p12_soc"
  [p10_current] -> Bus Creator12/10  "p10_current"
  PS-Simulink Converter123/1 -> [p1_current]
  [p12_cmd] -> Data Type Conversion11/1
  [p1_soc] -> Bus Creator10/1  "p1_soc"
  PS-Simulink Converter109/1 -> [p10_soc]
  [p7_soc] -> Bus Creator10/7  "p7_soc"
  [p1_cmd] -> Data Type Conversion/1
  Data Type Conversion/1 -> Delay19/1
  [p2_cmd] -> Data Type Conversion1/1
  Data Type Conversion1/1 -> Delay18/1
  [p3_cmd] -> Data Type Conversion2/1
  Data Type Conversion2/1 -> Delay17/1
  [p4_cmd] -> Data Type Conversion3/1
  Data Type Conversion3/1 -> Delay16/1
  PS-Simulink Converter62/1 -> [pack_voltage]
  Step2/1 -> Simulink-PS Converter22/1
  Step3/1 -> Simulink-PS Converter23/1
  Gain2/1 -> Simulink-PS Converter16/1
  Data Type Conversion4/1 -> Delay23/1
  Data Type Conversion5/1 -> Delay22/1
  Data Type Conversion6/1 -> Delay21/1
  Data Type Conversion7/1 -> Delay20/1
  Data Type Conversion8/1 -> Delay12/1
  Data Type Conversion9/1 -> Delay13/1
  Data Type Conversion10/1 -> Delay14/1
  Data Type Conversion11/1 -> Delay15/1
  Bus Creator12/1 -> Scope1/4
  Bus Creator10/1 -> Scope1/3
  Bus Creator3/1 -> Scope2/3
  PS-Simulink Converter196/1 -> Goto219/1
  From250/1 -> Bus Creator3/2  "p2_soc"
  From133/1 -> Bus Creator14/9  "p9_current"
  From254/1 -> Bus Creator14/2  "p2_current"
  PS-Simulink Converter90/1 -> Goto108/1
  Data Type Conversion17/1 -> Delay11/1
  PS-Simulink Converter191/1 -> Goto225/1
  Data Type Conversion13/1 -> Delay9/1
  PS-Simulink Converter93/1 -> Goto123/1
  PS-Simulink Converter198/1 -> Goto224/1
  PS-Simulink Converter193/1 -> Goto216/1
  PS-Simulink Converter66/1 -> Goto104/1
  From180/1 -> Bus Creator3/1  "p1_soc"
  From117/1 -> Bus Creator14/7  "p7_current"
  PS-Simulink Converter119/1 -> Goto191/1
  From93/1 -> Data Type Conversion19/1
  PS-Simulink Converter113/1 -> Goto198/1
  From146/1 -> Bus Creator3/9  "p9_soc"
  Data Type Conversion12/1 -> Delay8/1
  PS-Simulink Converter118/1 -> Goto204/1
  From179/1 -> Bus Creator14/1  "p1_current"
  From94/1 -> Data Type Conversion20/1
  PS-Simulink Converter188/1 -> Goto208/1
  From136/1 -> Bus Creator14/11  "p11_current"
  From124/1 -> Bus Creator3/8  "p8_soc"
  From181/1 -> balancing2/1(pack_current)  "pack_current"
  From149/1 -> Bus Creator3/11  "p11_soc"
  Data Type Conversion22/1 -> Delay/1
  PS-Simulink Converter186/1 -> Goto215/1
  From252/1 -> Data Type Conversion13/1
  From159/1 -> Bus Creator13/11  "p11_volt"
  PS-Simulink Converter70/1 -> Goto110/1
  From255/1 -> Data Type Conversion17/1
  PS-Simulink Converter121/1 -> Goto207/1
  PS-Simulink Converter103/1 -> Goto192/1
  PS-Simulink Converter98/1 -> Goto189/1
  PS-Simulink Converter68/1 -> Goto109/1
  Constant5/1 -> Simulink-PS Converter46/1
  From109/1 -> Bus Creator14/5  "p5_current"
  From104/1 -> Bus Creator13/2  "p2_volt"
  From99/1 -> Bus Creator13/1  "p1_volt"
  PS-Simulink Converter115/1 -> Goto201/1
  From253/1 -> Data Type Conversion16/1
  From257/1 -> Data Type Conversion23/1
  PS-Simulink Converter82/1 -> Goto118/1
  From87/1 -> Data Type Conversion18/1
  PS-Simulink Converter192/1 -> Goto212/1
  From154/1 -> Bus Creator13/9  "p9_volt"
  PS-Simulink Converter111/1 -> Goto197/1
  PS-Simulink Converter106/1 -> Goto195/1
  Data Type Conversion16/1 -> Delay10/1
  PS-Simulink Converter76/1 -> Goto112/1
  From95/1 -> Data Type Conversion21/1
  From158/1 -> Bus Creator13/10  "p10_volt"
  From148/1 -> Bus Creator3/10  "p10_soc"
  PS-Simulink Converter87/1 -> Goto119/1
  Data Type Conversion18/1 -> Delay4/1
  PS-Simulink Converter72/1 -> Goto196/1
  PS-Simulink Converter189/1 -> Goto213/1
  From129/1 -> Data Type Conversion15/1
  From106/1 -> Bus Creator13/3  "p3_volt"
  Data Type Conversion14/1 -> Delay2/1
  From135/1 -> Bus Creator14/10  "p10_current"
  Data Type Conversion20/1 -> Delay6/1
  Data Type Conversion21/1 -> Delay7/1
  From111/1 -> Bus Creator14/6  "p6_current"
  PS-Simulink Converter102/1 -> Goto203/1
  Data Type Conversion15/1 -> Delay3/1
  Step7/1 -> Simulink-PS Converter53/1
  Data Type Conversion23/1 -> Delay1/1
  From142/1 -> Bus Creator14/12  "p12_current"
  PS-Simulink Converter88/1 -> Goto122/1
  PS-Simulink Converter195/1 -> Goto222/1
  Bus Creator14/1 -> Scope2/4
  balancing2/1(cell_bal_cmd) -> Demux5/1, Scope2/1
  From176/1 -> Bus Creator14/8  "p8_current"
  PS-Simulink Converter79/1 -> Goto98/1
  PS-Simulink Converter99/1 -> Goto190/1
  From152/1 -> Bus Creator3/12  "p12_soc"
  From107/1 -> Bus Creator13/4  "p4_volt"
  PS-Simulink Converter199/1 -> Goto221/1
  From249/1 -> Bus Creator14/3  "p3_current"
  PS-Simulink Converter85/1 -> Goto115/1
  Step6/1 -> Simulink-PS Converter52/1
  From96/1 -> Bus Creator14/4  "p4_current"
  From120/1 -> Data Type Conversion14/1
  From123/1 -> Bus Creator3/7  "p7_soc"
  PS-Simulink Converter65/1 -> Goto103/1
  From126/1 -> Bus Creator13/7  "p7_volt"
  PS-Simulink Converter187/1 -> Goto205/1
  From256/1 -> Data Type Conversion22/1
  From97/1 -> Bus Creator3/3  "p3_soc"
  Bus Creator13/1 -> balancing2/2(cell_voltages), Scope2/2
  Data Type Conversion19/1 -> Delay5/1
  From125/1 -> Bus Creator13/6  "p6_volt"
  From131/1 -> Bus Creator13/8  "p8_volt"
  PS-Simulink Converter194/1 -> Goto223/1
  PS-Simulink Converter190/1 -> Goto209/1
  From165/1 -> Bus Creator13/12  "p12_volt"
  From118/1 -> Bus Creator3/5  "p5_soc"
  PS-Simulink Converter197/1 -> Goto96/1
  From251/1 -> Data Type Conversion12/1
  From122/1 -> Bus Creator3/6  "p6_soc"
  From177/1 -> Bus Creator13/5  "p5_volt"
  From98/1 -> Bus Creator3/4  "p4_soc"
  Delay/1 -> Simulink-PS Converter48/1
  Delay1/1 -> Simulink-PS Converter50/1
  Delay2/1 -> Simulink-PS Converter49/1
  Delay3/1 -> Simulink-PS Converter51/1
  Delay4/1 -> Simulink-PS Converter57/1
  Delay5/1 -> Simulink-PS Converter58/1
  Delay6/1 -> Simulink-PS Converter59/1
  Delay7/1 -> Simulink-PS Converter47/1
  Delay8/1 -> Simulink-PS Converter45/1
  Delay9/1 -> Simulink-PS Converter55/1
  Delay10/1 -> Simulink-PS Converter54/1
  Delay11/1 -> Simulink-PS Converter56/1
  Delay12/1 -> Simulink-PS Converter18/1
  Delay13/1 -> Simulink-PS Converter20/1
  Delay14/1 -> Simulink-PS Converter19/1
  Delay15/1 -> Simulink-PS Converter21/1
  Delay16/1 -> Simulink-PS Converter26/1
  Delay17/1 -> Simulink-PS Converter24/1
  Delay18/1 -> Simulink-PS Converter25/1
  Delay19/1 -> Simulink-PS Converter15/1
  Delay20/1 -> Simulink-PS Converter17/1
  Delay21/1 -> Simulink-PS Converter29/1
  Delay22/1 -> Simulink-PS Converter28/1
  Delay23/1 -> Simulink-PS Converter27/1
  Data Type Conversion34/1 -> Delay24/1
  From296/1 -> Data Type Conversion24/1
  PS-Simulink Converter212/1 -> Goto238/1
  From277/1 -> Bus Creator17/9  "p9_current"
  From144/1 -> Data Type Conversion30/1
  Demux3/4 -> Goto250/1  "p4_cmd"
  Demux3/11 -> Goto268/1  "p11_cmd"
  From281/1 -> Bus Creator15/9  "p9_soc"
  Delay27/1 -> Simulink-PS Converter66/1
  From264/1 -> Bus Creator16/4  "p4_volt"
  From290/1 -> Bus Creator16/5  "p5_volt"
  Bus Creator17/1 -> Scope3/4
  From283/1 -> Bus Creator15/11  "p11_soc"
  From150/1 -> Data Type Conversion31/1
  Delay29/1 -> Simulink-PS Converter69/1
  From263/1 -> Bus Creator16/3  "p3_volt"
  From289/1 -> Bus Creator17/8  "p8_current"
  PS-Simulink Converter226/1 -> Goto258/1
  PS-Simulink Converter235/1 -> Goto226/1
  PS-Simulink Converter213/1 -> Goto239/1
  PS-Simulink Converter225/1 -> Goto255/1
  Step9/1 -> Simulink-PS Converter68/1
  Bus Creator15/1 -> Scope3/3
  PS-Simulink Converter211/1 -> Goto230/1
  From266/1 -> Bus Creator17/6  "p6_current"
  Delay31/1 -> Simulink-PS Converter60/1
  PS-Simulink Converter203/1 -> Goto232/1
  From286/1 -> Bus Creator16/10  "p10_volt"
  PS-Simulink Converter210/1 -> Goto237/1
  Delay33/1 -> Simulink-PS Converter74/1
  Demux3/6 -> Goto256/1  "p6_cmd"
  Demux3/5 -> Goto252/1  "p5_cmd"
  Data Type Conversion35/1 -> Delay25/1
  From261/1 -> Bus Creator16/1  "p1_volt"
  Delay34/1 -> Simulink-PS Converter73/1
  Data Type Conversion31/1 -> Delay34/1
  PS-Simulink Converter209/1 -> Goto236/1
  From270/1 -> Bus Creator15/6  "p6_soc"
  PS-Simulink Converter233/1 -> Goto272/1
  From285/1 -> Bus Creator16/9  "p9_volt"
  Data Type Conversion29/1 -> Delay28/1
  Data Type Conversion25/1 -> Delay30/1
  From282/1 -> Bus Creator15/10  "p10_soc"
  Data Type Conversion24/1 -> Delay31/1
  From156/1 -> Data Type Conversion32/1
  From292/1 -> Bus Creator15/1  "p1_soc"
  PS-Simulink Converter229/1 -> Goto275/1
  Data Type Conversion26/1 -> Delay26/1
  Demux3/10 -> Goto267/1  "p10_cmd"
  From291/1 -> Bus Creator17/1  "p1_current"
  PS-Simulink Converter214/1 -> Goto240/1
  PS-Simulink Converter218/1 -> Goto247/1
  From278/1 -> Bus Creator17/10  "p10_current"
  From258/1 -> Bus Creator17/4  "p4_current"
  Delay30/1 -> Simulink-PS Converter70/1
  PS-Simulink Converter216/1 -> Goto242/1
  From272/1 -> Bus Creator15/8  "p8_soc"
  From265/1 -> Bus Creator17/5  "p5_current"
  From267/1 -> Bus Creator17/7  "p7_current"
  From269/1 -> Data Type Conversion26/1
  From288/1 -> Bus Creator16/12  "p12_volt"
  PS-Simulink Converter208/1 -> Goto234/1
  Demux3/3 -> Goto249/1  "p3_cmd"
  PS-Simulink Converter236/1 -> Goto274/1
  PS-Simulink Converter217/1 -> Goto245/1
  From161/1 -> Data Type Conversion33/1
  Data Type Conversion30/1 -> Delay35/1
  From268/1 -> Bus Creator15/5  "p5_soc"
  From298/1 -> Data Type Conversion28/1
  From275/1 -> Data Type Conversion27/1
  PS-Simulink Converter201/1 -> Goto229/1
  From279/1 -> Bus Creator17/11  "p11_current"
  Demux3/1 -> Goto243/1  "p1_cmd"
  From295/1 -> Bus Creator15/2  "p2_soc"
  PS-Simulink Converter232/1 -> Goto273/1
  PS-Simulink Converter204/1 -> Goto246/1
  PS-Simulink Converter234/1 -> Goto269/1
  Delay35/1 -> Simulink-PS Converter72/1
  From284/1 -> Bus Creator15/12  "p12_soc"
  PS-Simulink Converter222/1 -> Goto241/1
  Data Type Conversion33/1 -> Delay32/1
  PS-Simulink Converter219/1 -> Goto248/1
  Delay24/1 -> Simulink-PS Converter63/1
  PS-Simulink Converter202/1 -> Goto231/1
  PS-Simulink Converter207/1 -> Goto235/1
  PS-Simulink Converter206/1 -> Goto227/1
  PS-Simulink Converter223/1 -> Goto257/1
  From262/1 -> Bus Creator16/2  "p2_volt"
  Demux3/7 -> Goto260/1  "p7_cmd"
  From280/1 -> Bus Creator17/12  "p12_current"
  Delay25/1 -> Simulink-PS Converter65/1
  From271/1 -> Bus Creator15/7  "p7_soc"
  Delay26/1 -> Simulink-PS Converter64/1
  From300/1 -> Data Type Conversion29/1
  PS-Simulink Converter205/1 -> Goto233/1
  From287/1 -> Bus Creator16/11  "p11_volt"
  PS-Simulink Converter237/1 -> Goto271/1
  From259/1 -> Bus Creator15/3  "p3_soc"
  Delay28/1 -> Simulink-PS Converter71/1
  PS-Simulink Converter231/1 -> Goto266/1
  From299/1 -> Bus Creator17/2  "p2_current"
  Data Type Conversion28/1 -> Delay29/1
  From294/1 -> Bus Creator17/3  "p3_current"
  PS-Simulink Converter227/1 -> Goto263/1
  From260/1 -> Bus Creator15/4  "p4_soc"
  From302/1 -> Data Type Conversion35/1
  From276/1 -> Bus Creator16/8  "p8_volt"
  PS-Simulink Converter220/1 -> Goto251/1
  PS-Simulink Converter221/1 -> Goto254/1
  PS-Simulink Converter224/1 -> Goto265/1
  Delay32/1 -> Simulink-PS Converter62/1
  From301/1 -> Data Type Conversion34/1
  Data Type Conversion32/1 -> Delay33/1
  Step8/1 -> Simulink-PS Converter67/1
  Switch1/1 -> Gain1/1
  Demux3/8 -> Goto261/1  "p8_cmd"
  PS-Simulink Converter228/1 -> Goto259/1
  Demux3/12 -> Goto270/1  "p12_cmd"
  PS-Simulink Converter215/1 -> Goto253/1
  From297/1 -> Data Type Conversion25/1
  Demux3/2 -> Goto244/1  "p2_cmd"
  From274/1 -> Bus Creator16/7  "p7_volt"
  Demux3/9 -> Goto264/1  "p9_cmd"
  From273/1 -> Bus Creator16/6  "p6_volt"
  Data Type Conversion27/1 -> Delay27/1
  PS-Simulink Converter230/1 -> Goto262/1
  PS-Simulink Converter200/1 -> Goto228/1
  From200/1 -> Bus Creator18/11  "p11_soc"
  From207/1 -> Bus Creator19/5  "p5_volt"
  Delay39/1 -> Simulink-PS Converter36/1
  PS-Simulink Converter159/1 -> Goto126/1
  From175/1 -> Bus Creator19/3  "p3_volt"
  From167/1 -> Data Type Conversion43/1
  From201/1 -> Bus Creator18/12  "p12_soc"
  Delay47/1 -> Simulink-PS Converter42/1
  PS-Simulink Converter158/1 -> Goto169/1
  PS-Simulink Converter156/1 -> Goto173/1
  Data Type Conversion42/1 -> Delay47/1
  From215/1 -> Data Type Conversion40/1
  PS-Simulink Converter141/1 -> Goto145/1
  From192/1 -> Data Type Conversion39/1
  PS-Simulink Converter125/1 -> Goto129/1
  PS-Simulink Converter132/1 -> Goto134/1
  PS-Simulink Converter160/1 -> Goto174/1
  From205/1 -> Bus Creator19/12  "p12_volt"
  Bus Creator19/1 -> Scope4/2, To File/1, balancing3/2(cell_voltages)
  PS-Simulink Converter140/1 -> Goto142/1
  From184/1 -> Bus Creator20/7  "p7_current"
  Delay42/1 -> Simulink-PS Converter40/1
  From189/1 -> Bus Creator18/8  "p8_soc"
  PS-Simulink Converter138/1 -> Goto140/1
  Data Type Conversion38/1 -> Delay38/1
  From185/1 -> Bus Creator18/5  "p5_soc"
  From170/1 -> Bus Creator20/4  "p4_current"
  PS-Simulink Converter128/1 -> Goto146/1
  From208/1 -> Bus Creator20/1  "p1_current"
  Data Type Conversion37/1 -> Delay42/1
  From199/1 -> Bus Creator18/10  "p10_soc"
  From202/1 -> Bus Creator19/9  "p9_volt"
  Data Type Conversion36/1 -> Delay43/1
  Delay46/1 -> Simulink-PS Converter43/1
  From173/1 -> Bus Creator19/1  "p1_volt"
  Data Type Conversion47/1 -> Delay37/1
  PS-Simulink Converter134/1 -> Goto137/1
  Delay45/1 -> Simulink-PS Converter44/1
  From194/1 -> Bus Creator20/9  "p9_current"
  PS-Simulink Converter124/1 -> Goto128/1
  PS-Simulink Converter154/1 -> Goto162/1
  PS-Simulink Converter139/1 -> Goto153/1
  From191/1 -> Bus Creator19/7  "p7_volt"
  From214/1 -> Data Type Conversion37/1
  PS-Simulink Converter150/1 -> Goto158/1
  Delay44/1 -> Simulink-PS Converter32/1
  Data Type Conversion44/1 -> Delay45/1
  PS-Simulink Converter148/1 -> Goto165/1
  From193/1 -> Bus Creator19/8  "p8_volt"
  PS-Simulink Converter145/1 -> Goto154/1
  From219/1 -> Data Type Conversion47/1
  From206/1 -> Bus Creator20/8  "p8_current"
  From216/1 -> Bus Creator20/2  "p2_current"
  PS-Simulink Converter151/1 -> Goto163/1
  balancing3/1(cell_bal_cmd) -> Demux4/1, Data Type Conversion48/1, Scope4/1
  From218/1 -> Data Type Conversion46/1
  From210/1 -> balancing3/1(pack_current)  "pack_current"
  From204/1 -> Bus Creator19/11  "p11_volt"
  PS-Simulink Converter161/1 -> Goto171/1
  Delay40/1 -> Simulink-PS Converter41/1
  PS-Simulink Converter155/1 -> Goto166/1
  From188/1 -> Bus Creator18/7  "p7_soc"
  PS-Simulink Converter129/1 -> Goto133/1
  From217/1 -> Data Type Conversion41/1
  Delay38/1 -> Simulink-PS Converter34/1
  From174/1 -> Bus Creator19/2  "p2_volt"
  Delay37/1 -> Simulink-PS Converter35/1
  PS-Simulink Converter147/1 -> Goto157/1
  From187/1 -> Bus Creator18/6  "p6_soc"
  PS-Simulink Converter131/1 -> Goto135/1
  Delay36/1 -> Simulink-PS Converter33/1
  Data Type Conversion45/1 -> Delay44/1
  PS-Simulink Converter130/1 -> Goto127/1
  PS-Simulink Converter126/1 -> Goto131/1
  From169/1 -> Data Type Conversion45/1
  PS-Simulink Converter133/1 -> Goto136/1
  Delay41/1 -> Simulink-PS Converter39/1
  From203/1 -> Bus Creator19/10  "p10_volt"
  PS-Simulink Converter127/1 -> Goto132/1
  Delay43/1 -> Simulink-PS Converter30/1
  PS-Simulink Converter135/1 -> Goto130/1
  Bus Creator18/1 -> Scope4/3
  PS-Simulink Converter149/1 -> Goto155/1
  Step5/1 -> Simulink-PS Converter38/1
  PS-Simulink Converter157/1 -> Goto172/1
  PS-Simulink Converter137/1 -> Goto139/1
  From197/1 -> Bus Creator20/12  "p12_current"
  From211/1 -> Bus Creator20/3  "p3_current"
  From213/1 -> Data Type Conversion36/1
  Data Type Conversion46/1 -> Delay36/1
  PS-Simulink Converter136/1 -> Goto138/1
  PS-Simulink Converter143/1 -> Goto148/1
  From186/1 -> Data Type Conversion38/1
  PS-Simulink Converter146/1 -> Goto141/1
  Data Type Conversion40/1 -> Delay41/1
  From212/1 -> Bus Creator18/2  "p2_soc"
  From171/1 -> Bus Creator18/3  "p3_soc"
  PS-Simulink Converter142/1 -> Goto147/1
  PS-Simulink Converter153/1 -> Goto175/1
  From190/1 -> Bus Creator19/6  "p6_volt"
  From196/1 -> Bus Creator20/11  "p11_current"
  PS-Simulink Converter144/1 -> Goto151/1
  From195/1 -> Bus Creator20/10  "p10_current"
  From198/1 -> Bus Creator18/9  "p9_soc"
  Data Type Conversion41/1 -> Delay40/1
  Data Type Conversion43/1 -> Delay46/1
  From182/1 -> Bus Creator20/5  "p5_current"
  PS-Simulink Converter152/1 -> Goto159/1
  From209/1 -> Bus Creator18/1  "p1_soc"
  From183/1 -> Bus Creator20/6  "p6_current"
  From172/1 -> Bus Creator18/4  "p4_soc"
  Bus Creator20/1 -> Scope4/4
  Data Type Conversion39/1 -> Delay39/1
  Step4/1 -> Simulink-PS Converter37/1
  From168/1 -> Data Type Conversion44/1
  From178/1 -> Bus Creator19/4  "p4_volt"
  From166/1 -> Data Type Conversion42/1
  Pulse Generator1/1 -> balancing3/Trigger
  Demux4/7 -> Goto7/1  "p7_cmd"
  Demux4/9 -> Goto9/1  "p9_cmd"
  Demux4/3 -> Goto3/1  "p3_cmd"
  Demux4/2 -> Goto2/1  "p2_cmd"
  Demux4/8 -> Goto8/1  "p8_cmd"
  Demux4/1 -> Goto1/1  "p1_cmd"
  Demux4/4 -> Goto4/1  "p4_cmd"
  Demux4/10 -> Goto10/1  "p10_cmd"
  Demux4/6 -> Goto6/1  "p6_cmd"
  Demux4/12 -> Goto12/1  "p12_cmd"
  Demux4/5 -> Goto5/1  "p5_cmd"
  Demux4/11 -> Goto11/1  "p11_cmd"
  Pulse Generator3/1 -> balancing2/Trigger
  Demux5/7 -> Goto19/1  "p7_cmd"
  Demux5/9 -> Goto21/1  "p9_cmd"
  Demux5/3 -> Goto15/1  "p3_cmd"
  Demux5/2 -> Goto14/1  "p2_cmd"
  Demux5/8 -> Goto20/1  "p8_cmd"
  Demux5/1 -> Goto13/1  "p1_cmd"
  Demux5/4 -> Goto16/1  "p4_cmd"
  Demux5/10 -> Goto22/1  "p10_cmd"
  Demux5/6 -> Goto18/1  "p6_cmd"
  Demux5/12 -> Goto24/1  "p12_cmd"
  Demux5/5 -> Goto17/1  "p5_cmd"
  Demux5/11 -> Goto23/1  "p11_cmd"
  Demux1/4 -> [p4_cmd]  "p4_cmd"
  Demux1/6 -> [p6_cmd]  "p6_cmd"
  Demux1/11 -> [p11_cmd]  "p11_cmd"
  Demux1/10 -> [p10_cmd]  "p10_cmd"
  Demux1/12 -> [p12_cmd]  "p12_cmd"
  Demux1/5 -> [p5_cmd]  "p5_cmd"
  Demux1/8 -> [p8_cmd]  "p8_cmd"
  Demux1/1 -> [p1_cmd]  "p1_cmd"
  Demux1/2 -> [p2_cmd]  "p2_cmd"
  Demux1/3 -> [p3_cmd]  "p3_cmd"
  Demux1/7 -> [p7_cmd]  "p7_cmd"
  Demux1/9 -> [p9_cmd]  "p9_cmd"
  Data Type Conversion48/1 -> To File1/1
  Gain/1 -> Simulink-PS Converter31/1
  From2/1 -> Scope/2  "pack_current"
  From/1 -> Scope/1  "pack_voltage"
  Switch/1 -> Gain/1
  Repeating Sequence/1 -> Switch/1
  Step1/1 -> Switch/2
  Constant/1 -> Switch/3
  Constant1/1 -> Switch1/3
  Step10/1 -> Switch1/2
  Repeating Sequence1/1 -> Switch1/1
  Data Type Conversion49/1 -> To File3/1
  Bus Creator16/1 -> Scope3/2, To File2/1, balancing5/2(cell_voltages)
  From3/1 -> balancing5/1(pack_current)  "pack_current"
  Pulse Generator5/1 -> balancing5/Trigger
  balancing5/1(cell_bal_cmd) -> Demux3/1, Scope3/1, Data Type Conversion49/1
  From5/1 -> Scope5/2  "pack_current"
  From4/1 -> Scope5/1  "pack_voltage"
  Gain1/1 -> Simulink-PS Converter61/1
  [pack_voltage] -> Scope6/1  "pack_voltage"
  [pack_current] -> Scope6/2  "pack_current"
  Data Type Conversion50/1 -> To File5/1
  balancing1/1(cell_bal_cmd) -> Scope1/1, Demux1/1, Data Type Conversion50/1
  [pack_current] -> balancing1/1(pack_current)  "pack_current"
  Bus Creator11/1 -> balancing1/2(cell_voltages), To File4/1, Scope1/2
  Pulse Generator2/1 -> balancing1/Trigger
  Repeating Sequence2/1 -> Switch2/1
  Step11/1 -> Switch2/2
  Constant2/1 -> Switch2/3
  Switch2/1 -> Gain2/1
  connections:
  Resistor25/RConn1 -- Current Sensor36/RConn2 -- Voltage Sensor15/LConn1 -- SPST Switch18/LConn2 -- Voltage Sensor24/RConn2 -- BOL TWAICE Cell Model Pair 9/RConn1
  Current Sensor25/RConn2 -- Resistor17/RConn1 -- BOL TWAICE Cell Model Pair 12/RConn1 -- Voltage Sensor17/RConn2
  Voltage Sensor17/LConn1 -- Current Sensor41/RConn2 -- Voltage Sensor16/RConn2 -- BOL TWAICE Cell Model Pair 11/RConn1 -- Resistor15/RConn1 -- SPST Switch19/LConn2
  Voltage Sensor18/LConn1 -- SPST Switch25/LConn2 -- Current Sensor29/RConn2 -- Resistor21/RConn1 -- Voltage Sensor25/RConn2 -- BOL TWAICE Cell Model Pair 5/RConn1
  Voltage Sensor20/LConn1 -- SPST Switch27/LConn2 -- Current Sensor32/RConn2 -- Voltage Sensor22/RConn2 -- Resistor23/RConn1 -- BOL TWAICE Cell Model Pair 7/RConn1
  Voltage Sensor18/RConn2 -- Resistor22/RConn1 -- BOL TWAICE Cell Model Pair 6/RConn1 -- SPST Switch26/LConn2 -- Current Sensor30/RConn2 -- Voltage Sensor22/LConn1
  Voltage Sensor15/RConn2 -- BOL TWAICE Cell Model Pair 10/RConn1 -- Resistor16/RConn1 -- Voltage Sensor16/LConn1 -- Current Sensor39/RConn2 -- SPST Switch17/LConn2
  Resistor13/RConn1 -- SPST Switch20/LConn2 -- Voltage Sensor14/LConn1 -- Current Sensor43/RConn2 -- Voltage Sensor13/RConn2 -- BOL TWAICE Cell Model Pair 1/RConn1
  SPST Switch15/LConn2 -- Voltage Sensor21/LConn1 -- Current Sensor45/RConn2 -- Resistor18/RConn1 -- BOL TWAICE Cell Model Pair 2/RConn1 -- Voltage Sensor14/RConn2
  Voltage Sensor24/LConn1 -- Current Sensor34/RConn2 -- BOL TWAICE Cell Model Pair 8/RConn1 -- Resistor24/RConn1 -- Voltage Sensor20/RConn2 -- SPST Switch16/LConn2
  Current Sensor27/RConn2 -- Voltage Sensor25/LConn1 -- SPST Switch24/LConn2 -- BOL TWAICE Cell Model Pair 4/RConn1 -- Voltage Sensor23/RConn2 -- Resistor19/RConn1
  Voltage Sensor23/LConn1 -- Current Sensor47/RConn2 -- Voltage Sensor21/RConn2 -- BOL TWAICE Cell Model Pair 3/RConn1 -- Resistor14/RConn1 -- SPST Switch21/LConn2
  Resistor23/LConn1 -- SPST Switch26/RConn1
  Current Sensor30/LConn1 -- BOL TWAICE Cell Model Pair 7/LConn1
  Simulink-PS Converter20/RConn1 -- SPST Switch18/LConn1
  Resistor22/LConn1 -- SPST Switch25/RConn1
  PS-Simulink Converter120/LConn1 -- Current Sensor34/RConn1
  Voltage Sensor16/RConn1 -- PS-Simulink Converter105/LConn1
  Voltage Sensor21/RConn1 -- PS-Simulink Converter71/LConn1
  Current Sensor29/LConn1 -- BOL TWAICE Cell Model Pair 6/LConn1
  Simulink-PS Converter28/RConn1 -- SPST Switch25/LConn1
  Resistor17/LConn1 -- SPST Switch19/RConn1
  Resistor15/LConn1 -- SPST Switch17/RConn1
  Resistor25/LConn1 -- SPST Switch16/RConn1
  Resistor19/LConn1 -- SPST Switch21/RConn1
  Simulink-PS Converter19/RConn1 -- SPST Switch17/LConn1
  BOL TWAICE Cell Model Pair 11/LConn2 -- PS-Simulink Converter104/LConn1
  BOL TWAICE Cell Model Pair 9/LConn2 -- PS-Simulink Converter100/LConn1
  PS-Simulink Converter108/LConn1 -- Current Sensor39/RConn1
  Simulink-PS Converter21/RConn1 -- SPST Switch19/LConn1
  Current Sensor41/LConn1 -- BOL TWAICE Cell Model Pair 12/LConn1
  Current Sensor34/LConn1 -- BOL TWAICE Cell Model Pair 9/LConn1
  Resistor16/LConn1 -- SPST Switch18/RConn1
  BOL TWAICE Cell Model Pair 10/LConn2 -- PS-Simulink Converter109/LConn1
  BOL TWAICE Cell Model Pair 2/LConn2 -- PS-Simulink Converter74/LConn1
  PS-Simulink Converter81/LConn1 -- BOL TWAICE Cell Model Pair 5/LConn2
  Simulink-PS Converter18/RConn1 -- SPST Switch16/LConn1
  Resistor21/LConn1 -- SPST Switch24/RConn1
  Current Sensor27/LConn1 -- BOL TWAICE Cell Model Pair 5/LConn1
  PS-Simulink Converter91/LConn1 -- BOL TWAICE Cell Model Pair 8/LConn2
  PS-Simulink Converter92/LConn1 -- BOL TWAICE Cell Model Pair 7/LConn2
  BOL TWAICE Cell Model Pair 4/LConn2 -- PS-Simulink Converter78/LConn1
  PS-Simulink Converter80/LConn1 -- Voltage Sensor23/RConn1
  BOL TWAICE Cell Model Pair 4/LConn1 -- Current Sensor47/LConn1
  Voltage Sensor22/RConn1 -- PS-Simulink Converter95/LConn1
  PS-Simulink Converter112/LConn1 -- BOL TWAICE Cell Model Pair 12/LConn2
  BOL TWAICE Cell Model Pair 8/LConn1 -- Current Sensor32/LConn1
  PS-Simulink Converter117/LConn1 -- Voltage Sensor15/RConn1
  PS-Simulink Converter94/LConn1 -- Voltage Sensor20/RConn1
  Simulink-PS Converter15/RConn1 -- SPST Switch14/LConn1
  Current Sensor26/LConn1 -- BOL TWAICE Cell Model Pair 1/LConn1
  Voltage Sensor13/RConn1 -- PS-Simulink Converter96/LConn1
  Resistor13/LConn1 -- SPST Switch14/RConn1
  PS-Simulink Converter64/LConn1 -- Current Sensor43/RConn1
  Simulink-PS Converter26/RConn1 -- SPST Switch21/LConn1
  Current Sensor29/RConn1 -- PS-Simulink Converter67/LConn1
  BOL TWAICE Cell Model Pair 3/LConn2 -- PS-Simulink Converter69/LConn1
  Current Sensor45/LConn1 -- BOL TWAICE Cell Model Pair 3/LConn1
  PS-Simulink Converter83/LConn1 -- Voltage Sensor18/RConn1
  Simulink-PS Converter27/RConn1 -- SPST Switch24/LConn1
  Simulink-PS Converter17/RConn1 -- SPST Switch27/LConn1
  Simulink-PS Converter29/RConn1 -- SPST Switch26/LConn1
  Voltage Sensor24/RConn1 -- PS-Simulink Converter116/LConn1
  Resistor24/LConn1 -- SPST Switch27/RConn1
  Simulink-PS Converter24/RConn1 -- SPST Switch15/LConn1
  Simulink-PS Converter25/RConn1 -- SPST Switch20/LConn1
  PS-Simulink Converter97/LConn1 -- Current Sensor30/RConn1
  Voltage Sensor25/RConn1 -- PS-Simulink Converter84/LConn1
  PS-Simulink Converter110/LConn1 -- Current Sensor41/RConn1
  Resistor18/LConn1 -- SPST Switch20/RConn1
  PS-Simulink Converter107/LConn1 -- Voltage Sensor14/RConn1
  Current Sensor32/RConn1 -- PS-Simulink Converter89/LConn1
  Current Sensor39/LConn1 -- BOL TWAICE Cell Model Pair 11/LConn1
  PS-Simulink Converter114/LConn1 -- Voltage Sensor17/RConn1
  BOL TWAICE Cell Model Pair 1/LConn2 -- PS-Simulink Converter63/LConn1
  PS-Simulink Converter123/LConn1 -- Current Sensor26/RConn1
  Current Sensor43/LConn1 -- BOL TWAICE Cell Model Pair 2/LConn1
  Resistor14/LConn1 -- SPST Switch15/RConn1
  Current Sensor36/LConn1 -- BOL TWAICE Cell Model Pair 10/LConn1
  PS-Simulink Converter86/LConn1 -- Current Sensor27/RConn1
  PS-Simulink Converter75/LConn1 -- Current Sensor47/RConn1
  Current Sensor25/RConn1 -- PS-Simulink Converter122/LConn1
  PS-Simulink Converter101/LConn1 -- Current Sensor36/RConn1
  PS-Simulink Converter73/LConn1 -- Current Sensor45/RConn1
  PS-Simulink Converter77/LConn1 -- BOL TWAICE Cell Model Pair 6/LConn2
  SPST Switch14/LConn2 -- Current Sensor26/RConn2 -- Voltage Sensor13/LConn1 -- SPST Switch23/LConn2 -- SPST Switch22/LConn2
  Diode1/LConn1 -- Controlled Current Source2/RConn2 -- Voltage Sensor39/LConn1 -- SPST Switch23/RConn1 -- Resistor20/RConn1
  MT42 Capacitance1/LConn1 -- Diode1/RConn1
  Simulink-PS Converter22/RConn1 -- SPST Switch23/LConn1
  Voltage Sensor39/RConn1 -- PS-Simulink Converter62/LConn1
  SPST Switch22/RConn1 -- Resistor20/LConn1
  Simulink-PS Converter23/RConn1 -- SPST Switch22/LConn1
  Voltage Sensor39/RConn2 -- Controlled Current Source2/LConn1 -- Solver Configuration/RConn1 -- Electrical Reference/LConn1 -- MT42 Capacitance1/RConn1 -- Current Sensor25/LConn1
  Simulink-PS Converter16/RConn1 -- Controlled Current Source2/RConn1
  Voltage Sensor49/RConn2 -- BOL HPPC Module Pair 9/RConn1 -- Resistor51/RConn1 -- Current Sensor42/RConn2 -- Voltage Sensor41/LConn1 -- SPST Switch46/LConn2
  SPST Switch52/LConn2 -- Current Sensor33/RConn2 -- BOL HPPC Module Pair 4/RConn1 -- Voltage Sensor48/RConn2 -- Resistor45/RConn1 -- Voltage Sensor50/LConn1
  Voltage Sensor19/RConn2 -- BOL HPPC Module Pair 1/RConn1 -- Resistor39/RConn1 -- SPST Switch48/LConn2 -- Voltage Sensor40/LConn1 -- Current Sensor48/RConn2
  Current Sensor28/LConn1 -- Voltage Sensor51/RConn2 -- Controlled Current Source4/LConn1 -- Solver Configuration2/RConn1 -- Electrical Reference1/LConn1 -- MT42 Capacitance3/RConn1
  Current Sensor37/RConn2 -- Resistor48/RConn1 -- Voltage Sensor44/RConn2 -- BOL HPPC Module Pair 6/RConn1 -- Voltage Sensor47/LConn1 -- SPST Switch54/LConn2
  SPST Switch45/LConn2 -- Voltage Sensor42/LConn1 -- Current Sensor44/RConn2 -- BOL HPPC Module Pair 10/RConn1 -- Voltage Sensor41/RConn2 -- Resistor42/RConn1
  SPST Switch47/LConn2 -- Voltage Sensor43/LConn1 -- Current Sensor46/RConn2 -- BOL HPPC Module Pair 11/RConn1 -- Voltage Sensor42/RConn2 -- Resistor41/RConn1
  SPST Switch49/LConn2 -- BOL HPPC Module Pair 3/RConn1 -- Voltage Sensor46/RConn2 -- Resistor40/RConn1 -- Voltage Sensor48/LConn1 -- Current Sensor75/RConn2
  SPST Switch50/LConn2 -- SPST Switch51/LConn2 -- SPST Switch42/LConn2 -- Current Sensor31/RConn2 -- Voltage Sensor19/LConn1
  Voltage Sensor40/RConn2 -- BOL HPPC Module Pair 2/RConn1 -- SPST Switch43/LConn2 -- Voltage Sensor46/LConn1 -- Current Sensor49/RConn2 -- Resistor44/RConn1
  Voltage Sensor50/RConn2 -- BOL HPPC Module Pair 5/RConn1 -- Resistor47/RConn1 -- Voltage Sensor44/LConn1 -- SPST Switch53/LConn2 -- Current Sensor35/RConn2
  Resistor49/RConn1 -- BOL HPPC Module Pair 7/RConn1 -- Voltage Sensor45/LConn1 -- SPST Switch55/LConn2 -- Current Sensor38/RConn2 -- Voltage Sensor47/RConn2
  Voltage Sensor43/RConn2 -- BOL HPPC Module Pair 12/RConn1 -- Current Sensor28/RConn2 -- Resistor43/RConn1
  SPST Switch51/RConn1 -- Diode3/LConn1 -- Controlled Current Source4/RConn2 -- Resistor46/RConn1 -- Voltage Sensor51/LConn1
  Resistor50/RConn1 -- BOL HPPC Module Pair 8/RConn1 -- Voltage Sensor45/RConn2 -- Voltage Sensor49/LConn1 -- Current Sensor40/RConn2 -- SPST Switch44/LConn2
  Simulink-PS Converter56/RConn1 -- SPST Switch49/LConn1
  BOL HPPC Module Pair 10/LConn2 -- PS-Simulink Converter79/LConn1
  MT42 Capacitance3/LConn1 -- Diode3/RConn1
  Resistor44/LConn1 -- SPST Switch48/RConn1
  PS-Simulink Converter106/LConn1 -- Current Sensor48/RConn1
  Resistor45/LConn1 -- SPST Switch49/RConn1
  BOL HPPC Module Pair 5/LConn2 -- PS-Simulink Converter189/LConn1
  Simulink-PS Converter55/RConn1 -- SPST Switch48/LConn1
  SPST Switch50/RConn1 -- Resistor46/LConn1
  Resistor48/LConn1 -- SPST Switch53/RConn1
  Simulink-PS Converter58/RConn1 -- SPST Switch53/LConn1
  PS-Simulink Converter66/LConn1 -- Current Sensor42/RConn1
  Simulink-PS Converter46/RConn1 -- Controlled Current Source4/RConn1
  Simulink-PS Converter50/RConn1 -- SPST Switch46/LConn1
  Voltage Sensor47/RConn1 -- PS-Simulink Converter197/LConn1
  BOL HPPC Module Pair 4/LConn1 -- Current Sensor75/LConn1
  PS-Simulink Converter99/LConn1 -- Current Sensor31/RConn1
  PS-Simulink Converter90/LConn1 -- Voltage Sensor41/RConn1
  Current Sensor35/RConn1 -- PS-Simulink Converter111/LConn1
  Simulink-PS Converter59/RConn1 -- SPST Switch54/LConn1
  PS-Simulink Converter199/LConn1 -- Current Sensor37/RConn1
  Voltage Sensor50/RConn1 -- PS-Simulink Converter191/LConn1
  BOL HPPC Module Pair 2/LConn1 -- Current Sensor48/LConn1
  BOL HPPC Module Pair 7/LConn1 -- Current Sensor37/LConn1
  PS-Simulink Converter188/LConn1 -- Voltage Sensor48/RConn1
  BOL HPPC Module Pair 10/LConn1 -- Current Sensor42/LConn1
  BOL HPPC Module Pair 7/LConn2 -- PS-Simulink Converter195/LConn1
  PS-Simulink Converter190/LConn1 -- Voltage Sensor44/RConn1
  Current Sensor38/LConn1 -- BOL HPPC Module Pair 8/LConn1
  BOL HPPC Module Pair 9/LConn2 -- PS-Simulink Converter65/LConn1
  PS-Simulink Converter93/LConn1 -- Current Sensor40/RConn1
  BOL HPPC Module Pair 9/LConn1 -- Current Sensor40/LConn1
  BOL HPPC Module Pair 6/LConn1 -- Current Sensor35/LConn1
  Simulink-PS Converter51/RConn1 -- SPST Switch47/LConn1
  Simulink-PS Converter47/RConn1 -- SPST Switch55/LConn1
  Voltage Sensor42/RConn1 -- PS-Simulink Converter70/LConn1
  Current Sensor28/RConn1 -- PS-Simulink Converter98/LConn1
  BOL HPPC Module Pair 3/LConn1 -- Current Sensor49/LConn1
  Voltage Sensor49/RConn1 -- PS-Simulink Converter88/LConn1
  Resistor39/LConn1 -- SPST Switch42/RConn1
  BOL HPPC Module Pair 3/LConn2 -- PS-Simulink Converter113/LConn1
  BOL HPPC Module Pair 1/LConn1 -- Current Sensor31/LConn1
  Simulink-PS Converter48/RConn1 -- SPST Switch44/LConn1
  Resistor41/LConn1 -- SPST Switch45/RConn1
  Resistor42/LConn1 -- SPST Switch46/RConn1
  Resistor47/LConn1 -- SPST Switch52/RConn1
  Simulink-PS Converter57/RConn1 -- SPST Switch52/LConn1
  Simulink-PS Converter49/RConn1 -- SPST Switch45/LConn1
  BOL HPPC Module Pair 4/LConn2 -- PS-Simulink Converter187/LConn1
  PS-Simulink Converter118/LConn1 -- Current Sensor49/RConn1
  BOL HPPC Module Pair 11/LConn2 -- PS-Simulink Converter68/LConn1
  Simulink-PS Converter54/RConn1 -- SPST Switch43/LConn1
  BOL HPPC Module Pair 12/LConn2 -- PS-Simulink Converter85/LConn1
  PS-Simulink Converter87/LConn1 -- Voltage Sensor43/RConn1
  Resistor50/LConn1 -- SPST Switch55/RConn1
  PS-Simulink Converter76/LConn1 -- Current Sensor44/RConn1
  PS-Simulink Converter192/LConn1 -- Current Sensor33/RConn1
  PS-Simulink Converter82/LConn1 -- Current Sensor46/RConn1
  BOL HPPC Module Pair 5/LConn1 -- Current Sensor33/LConn1
  Voltage Sensor51/RConn1 -- PS-Simulink Converter102/LConn1
  PS-Simulink Converter196/LConn1 -- Voltage Sensor45/RConn1
  BOL HPPC Module Pair 6/LConn2 -- PS-Simulink Converter186/LConn1
  Simulink-PS Converter53/RConn1 -- SPST Switch50/LConn1
  BOL HPPC Module Pair 11/LConn1 -- Current Sensor44/LConn1
  BOL HPPC Module Pair 1/LConn2 -- PS-Simulink Converter103/LConn1
  Voltage Sensor19/RConn1 -- PS-Simulink Converter198/LConn1
  Resistor49/LConn1 -- SPST Switch54/RConn1
  BOL HPPC Module Pair 12/LConn1 -- Current Sensor46/LConn1
  Current Sensor38/RConn1 -- PS-Simulink Converter193/LConn1
  BOL HPPC Module Pair 8/LConn2 -- PS-Simulink Converter194/LConn1
  PS-Simulink Converter72/LConn1 -- Voltage Sensor40/RConn1
  Simulink-PS Converter52/RConn1 -- SPST Switch51/LConn1
  Resistor51/LConn1 -- SPST Switch44/RConn1
  Simulink-PS Converter45/RConn1 -- SPST Switch42/LConn1
  Voltage Sensor46/RConn1 -- PS-Simulink Converter115/LConn1
  Resistor40/LConn1 -- SPST Switch43/RConn1
  Resistor43/LConn1 -- SPST Switch47/RConn1
  BOL HPPC Module Pair 2/LConn2 -- PS-Simulink Converter119/LConn1
  PS-Simulink Converter121/LConn1 -- Current Sensor75/RConn1
  Current Sensor76/LConn1 -- Voltage Sensor64/RConn2 -- Controlled Current Source5/LConn1 -- Solver Configuration4/RConn1 -- Electrical Reference4/LConn1 -- MT42 Capacitance4/RConn1
  SPST Switch59/LConn2 -- EOL TWAICE Cell Model Pair 10/RConn1 -- Voltage Sensor54/RConn2 -- Resistor55/RConn1 -- Voltage Sensor55/LConn1 -- Current Sensor84/RConn2
  Current Sensor79/RConn2 -- Voltage Sensor57/LConn1 -- EOL TWAICE Cell Model Pair 5/RConn1 -- Resistor60/RConn1 -- Voltage Sensor63/RConn2 -- SPST Switch67/LConn2
  Current Sensor86/RConn2 -- Resistor52/RConn1 -- EOL TWAICE Cell Model Pair 1/RConn1 -- Voltage Sensor52/RConn2 -- SPST Switch62/LConn2 -- Voltage Sensor53/LConn1
  SPST Switch66/LConn2 -- Current Sensor78/RConn2 -- EOL TWAICE Cell Model Pair 4/RConn1 -- Voltage Sensor61/RConn2 -- Resistor58/RConn1 -- Voltage Sensor63/LConn1
  Resistor54/RConn1 -- Voltage Sensor56/LConn1 -- Current Sensor85/RConn2 -- SPST Switch61/LConn2 -- EOL TWAICE Cell Model Pair 11/RConn1 -- Voltage Sensor55/RConn2
  Voltage Sensor58/RConn2 -- Voltage Sensor62/LConn1 -- Current Sensor82/RConn2 -- SPST Switch58/LConn2 -- EOL TWAICE Cell Model Pair 8/RConn1 -- Resistor63/RConn1
  SPST Switch65/RConn1 -- Diode4/LConn1 -- Controlled Current Source5/RConn2 -- Resistor59/RConn1 -- Voltage Sensor64/LConn1
  Voltage Sensor56/RConn2 -- EOL TWAICE Cell Model Pair 12/RConn1 -- Resistor56/RConn1 -- Current Sensor76/RConn2
  SPST Switch63/LConn2 -- EOL TWAICE Cell Model Pair 3/RConn1 -- Voltage Sensor59/RConn2 -- Resistor53/RConn1 -- Voltage Sensor61/LConn1 -- Current Sensor88/RConn2
  Resistor62/RConn1 -- EOL TWAICE Cell Model Pair 7/RConn1 -- Voltage Sensor58/LConn1 -- SPST Switch69/LConn2 -- Current Sensor81/RConn2 -- Voltage Sensor60/RConn2
  Current Sensor80/RConn2 -- EOL TWAICE Cell Model Pair 6/RConn1 -- Voltage Sensor57/RConn2 -- Resistor61/RConn1 -- Voltage Sensor60/LConn1 -- SPST Switch68/LConn2
  SPST Switch64/LConn2 -- SPST Switch56/LConn2 -- Current Sensor77/RConn2 -- Voltage Sensor52/LConn1 -- SPST Switch65/LConn2
  Voltage Sensor62/RConn2 -- EOL TWAICE Cell Model Pair 9/RConn1 -- Resistor64/RConn1 -- Current Sensor83/RConn2 -- Voltage Sensor54/LConn1 -- SPST Switch60/LConn2
  Voltage Sensor53/RConn2 -- EOL TWAICE Cell Model Pair 2/RConn1 -- Resistor57/RConn1 -- SPST Switch57/LConn2 -- Voltage Sensor59/LConn1 -- Current Sensor87/RConn2
  Simulink-PS Converter63/RConn1 -- SPST Switch58/LConn1
  Resistor57/LConn1 -- SPST Switch62/RConn1
  Resistor56/LConn1 -- SPST Switch61/RConn1
  PS-Simulink Converter223/LConn1 -- Current Sensor88/RConn1
  Simulink-PS Converter61/RConn1 -- Controlled Current Source5/RConn1
  EOL TWAICE Cell Model Pair 12/LConn1 -- Current Sensor85/LConn1
  PS-Simulink Converter201/LConn1 -- Current Sensor83/RConn1
  Simulink-PS Converter60/RConn1 -- SPST Switch56/LConn1
  Current Sensor79/LConn1 -- EOL TWAICE Cell Model Pair 6/LConn1
  PS-Simulink Converter230/LConn1 -- Current Sensor78/RConn1
  Current Sensor80/LConn1 -- EOL TWAICE Cell Model Pair 7/LConn1
  PS-Simulink Converter205/LConn1 -- Current Sensor84/RConn1
  Voltage Sensor64/RConn1 -- PS-Simulink Converter215/LConn1
  Current Sensor79/RConn1 -- PS-Simulink Converter218/LConn1
  PS-Simulink Converter217/LConn1 -- Current Sensor86/RConn1
  Current Sensor81/RConn1 -- PS-Simulink Converter231/LConn1
  PS-Simulink Converter211/LConn1 -- Voltage Sensor54/RConn1
  EOL TWAICE Cell Model Pair 9/LConn2 -- PS-Simulink Converter200/LConn1
  PS-Simulink Converter234/LConn1 -- Voltage Sensor58/RConn1
  PS-Simulink Converter207/LConn1 -- Current Sensor85/RConn1
  Voltage Sensor63/RConn1 -- PS-Simulink Converter229/LConn1
  EOL TWAICE Cell Model Pair 3/LConn1 -- Current Sensor87/LConn1
  Voltage Sensor62/RConn1 -- PS-Simulink Converter210/LConn1
  Simulink-PS Converter73/RConn1 -- SPST Switch67/LConn1
  Resistor53/LConn1 -- SPST Switch57/RConn1
  Simulink-PS Converter71/RConn1 -- SPST Switch63/LConn1
  Simulink-PS Converter70/RConn1 -- SPST Switch62/LConn1
  Current Sensor78/LConn1 -- EOL TWAICE Cell Model Pair 5/LConn1
  EOL TWAICE Cell Model Pair 9/LConn1 -- Current Sensor82/LConn1
  PS-Simulink Converter221/LConn1 -- Current Sensor87/RConn1
  Simulink-PS Converter72/RConn1 -- SPST Switch66/LConn1
  Current Sensor76/RConn1 -- PS-Simulink Converter213/LConn1
  EOL TWAICE Cell Model Pair 2/LConn2 -- PS-Simulink Converter222/LConn1
  Simulink-PS Converter66/RConn1 -- SPST Switch61/LConn1
  Current Sensor83/LConn1 -- EOL TWAICE Cell Model Pair 10/LConn1
  Simulink-PS Converter68/RConn1 -- SPST Switch64/LConn1
  Resistor54/LConn1 -- SPST Switch59/RConn1
  MT42 Capacitance4/LConn1 -- Diode4/RConn1
  Resistor60/LConn1 -- SPST Switch66/RConn1
  PS-Simulink Converter226/LConn1 -- Voltage Sensor61/RConn1
  PS-Simulink Converter202/LConn1 -- EOL TWAICE Cell Model Pair 11/LConn2
  PS-Simulink Converter204/LConn1 -- Voltage Sensor53/RConn1
  Resistor55/LConn1 -- SPST Switch60/RConn1
  Simulink-PS Converter67/RConn1 -- SPST Switch65/LConn1
  Resistor62/LConn1 -- SPST Switch68/RConn1
  EOL TWAICE Cell Model Pair 8/LConn2 -- PS-Simulink Converter232/LConn1
  EOL TWAICE Cell Model Pair 5/LConn2 -- PS-Simulink Converter227/LConn1
  EOL TWAICE Cell Model Pair 12/LConn2 -- PS-Simulink Converter208/LConn1
  EOL TWAICE Cell Model Pair 8/LConn1 -- Current Sensor81/LConn1
  EOL TWAICE Cell Model Pair 7/LConn2 -- PS-Simulink Converter233/LConn1
  PS-Simulink Converter225/LConn1 -- EOL TWAICE Cell Model Pair 4/LConn2
  PS-Simulink Converter214/LConn1 -- Current Sensor77/RConn1
  Current Sensor77/LConn1 -- EOL TWAICE Cell Model Pair 1/LConn1
  PS-Simulink Converter228/LConn1 -- Voltage Sensor57/RConn1
  SPST Switch64/RConn1 -- Resistor59/LConn1
  Simulink-PS Converter65/RConn1 -- SPST Switch60/LConn1
  EOL TWAICE Cell Model Pair 6/LConn2 -- PS-Simulink Converter224/LConn1
  Resistor58/LConn1 -- SPST Switch63/RConn1
  PS-Simulink Converter209/LConn1 -- Voltage Sensor56/RConn1
  Simulink-PS Converter62/RConn1 -- SPST Switch69/LConn1
  Voltage Sensor59/RConn1 -- PS-Simulink Converter220/LConn1
  Resistor61/LConn1 -- SPST Switch67/RConn1
  Voltage Sensor55/RConn1 -- PS-Simulink Converter203/LConn1
  Resistor64/LConn1 -- SPST Switch58/RConn1
  EOL TWAICE Cell Model Pair 2/LConn1 -- Current Sensor86/LConn1
  EOL TWAICE Cell Model Pair 10/LConn2 -- PS-Simulink Converter206/LConn1
  EOL TWAICE Cell Model Pair 1/LConn2 -- PS-Simulink Converter216/LConn1
  PS-Simulink Converter219/LConn1 -- EOL TWAICE Cell Model Pair 3/LConn2
  Current Sensor88/LConn1 -- EOL TWAICE Cell Model Pair 4/LConn1
  Simulink-PS Converter74/RConn1 -- SPST Switch68/LConn1
  Voltage Sensor52/RConn1 -- PS-Simulink Converter236/LConn1
  Voltage Sensor60/RConn1 -- PS-Simulink Converter235/LConn1
  Simulink-PS Converter69/RConn1 -- SPST Switch57/LConn1
  Simulink-PS Converter64/RConn1 -- SPST Switch59/LConn1
  Resistor52/LConn1 -- SPST Switch56/RConn1
  PS-Simulink Converter237/LConn1 -- Current Sensor80/RConn1
  Resistor63/LConn1 -- SPST Switch69/RConn1
  EOL TWAICE Cell Model Pair 11/LConn1 -- Current Sensor84/LConn1
  PS-Simulink Converter212/LConn1 -- Current Sensor82/RConn1
  Resistor36/RConn1 -- BOL TWAICE Cell Model Pair 19/RConn1 -- Voltage Sensor34/RConn2 -- Voltage Sensor32/LConn1 -- SPST Switch41/LConn2 -- Current Sensor55/RConn2
  SPST Switch37/RConn1 -- Voltage Sensor38/LConn1 -- Diode2/LConn1 -- Controlled Current Source3/RConn2 -- Resistor33/RConn1
  SPST Switch31/LConn2 -- Voltage Sensor29/LConn1 -- Current Sensor58/RConn2 -- EOL TWAICE Cell Model Pair 22/RConn1 -- Voltage Sensor28/RConn2 -- Resistor29/RConn1
  Current Sensor54/RConn2 -- SPST Switch40/LConn2 -- EOL TWAICE Cell Model Pair 18/RConn1 -- Voltage Sensor31/RConn2 -- Resistor35/RConn1 -- Voltage Sensor34/LConn1
  Current Sensor53/RConn2 -- SPST Switch39/LConn2 -- BOL TWAICE Cell Model Pair 17/RConn1 -- Resistor34/RConn1 -- Voltage Sensor37/RConn2 -- Voltage Sensor31/LConn1
  Current Sensor50/LConn1 -- Voltage Sensor38/RConn2 -- MT42 Capacitance2/RConn1 -- Electrical Reference2/LConn1 -- Controlled Current Source3/LConn1 -- Solver Configuration3/RConn1
  Resistor28/RConn1 -- BOL TWAICE Cell Model Pair 23/RConn1 -- Voltage Sensor29/RConn2 -- SPST Switch33/LConn2 -- Voltage Sensor30/LConn1 -- Current Sensor59/RConn2
  Voltage Sensor32/RConn2 -- EOL TWAICE Cell Model Pair 20/RConn1 -- Resistor37/RConn1 -- SPST Switch30/LConn2 -- Voltage Sensor36/LConn1 -- Current Sensor56/RConn2
  SPST Switch36/LConn2 -- SPST Switch37/LConn2 -- SPST Switch28/LConn2 -- Current Sensor51/RConn2 -- Voltage Sensor26/LConn1
  Current Sensor60/RConn2 -- Voltage Sensor27/LConn1 -- SPST Switch34/LConn2 -- Resistor26/RConn1 -- BOL TWAICE Cell Model Pair 13/RConn1 -- Voltage Sensor26/RConn2
  Voltage Sensor36/RConn2 -- BOL TWAICE Cell Model Pair 21/RConn1 -- Resistor38/RConn1 -- Current Sensor57/RConn2 -- Voltage Sensor28/LConn1 -- SPST Switch32/LConn2
  Current Sensor62/RConn2 -- Voltage Sensor35/LConn1 -- SPST Switch35/LConn2 -- BOL TWAICE Cell Model Pair 15/RConn1 -- Voltage Sensor33/RConn2 -- Resistor27/RConn1
  Voltage Sensor27/RConn2 -- EOL TWAICE Cell Model Pair 14/RConn1 -- Resistor31/RConn1 -- SPST Switch29/LConn2 -- Voltage Sensor33/LConn1 -- Current Sensor61/RConn2
  Current Sensor52/RConn2 -- Resistor32/RConn1 -- EOL TWAICE Cell Model Pair 16/RConn1 -- Voltage Sensor35/RConn2 -- Voltage Sensor37/LConn1 -- SPST Switch38/LConn2
  Current Sensor50/RConn2 -- Resistor30/RConn1 -- EOL TWAICE Cell Model Pair 24/RConn1 -- Voltage Sensor30/RConn2
  Current Sensor50/RConn1 -- PS-Simulink Converter137/LConn1
  Simulink-PS Converter32/RConn1 -- SPST Switch41/LConn1
  Current Sensor53/LConn1 -- EOL TWAICE Cell Model Pair 18/LConn1
  Simulink-PS Converter35/RConn1 -- SPST Switch32/LConn1
  Resistor34/LConn1 -- SPST Switch38/RConn1
  BOL TWAICE Cell Model Pair 17/LConn2 -- PS-Simulink Converter151/LConn1
  EOL TWAICE Cell Model Pair 14/LConn2 -- PS-Simulink Converter146/LConn1
  EOL TWAICE Cell Model Pair 18/LConn2 -- PS-Simulink Converter148/LConn1
  Resistor27/LConn1 -- SPST Switch29/RConn1
  EOL TWAICE Cell Model Pair 22/LConn2 -- PS-Simulink Converter130/LConn1
  Resistor29/LConn1 -- SPST Switch32/RConn1
  PS-Simulink Converter154/LConn1 -- Current Sensor52/RConn1
  Resistor32/LConn1 -- SPST Switch35/RConn1
  PS-Simulink Converter143/LConn1 -- BOL TWAICE Cell Model Pair 15/LConn2
  EOL TWAICE Cell Model Pair 20/LConn2 -- PS-Simulink Converter156/LConn1
  BOL TWAICE Cell Model Pair 13/LConn1 -- Current Sensor51/LConn1
  Current Sensor61/LConn1 -- BOL TWAICE Cell Model Pair 15/LConn1
  BOL TWAICE Cell Model Pair 19/LConn2 -- PS-Simulink Converter157/LConn1
  Voltage Sensor37/RConn1 -- PS-Simulink Converter153/LConn1
  PS-Simulink Converter136/LConn1 -- Current Sensor56/RConn1
  PS-Simulink Converter131/LConn1 -- Current Sensor59/RConn1
  Simulink-PS Converter34/RConn1 -- SPST Switch31/LConn1
  Simulink-PS Converter40/RConn1 -- SPST Switch34/LConn1
  BOL TWAICE Cell Model Pair 21/LConn2 -- PS-Simulink Converter124/LConn1
  Resistor37/LConn1 -- SPST Switch41/RConn1
  PS-Simulink Converter161/LConn1 -- Current Sensor54/RConn1
  Resistor26/LConn1 -- SPST Switch28/RConn1
  BOL TWAICE Cell Model Pair 23/LConn1 -- Current Sensor58/LConn1
  Simulink-PS Converter41/RConn1 -- SPST Switch35/LConn1
  PS-Simulink Converter150/LConn1 -- Voltage Sensor35/RConn1
  Simulink-PS Converter44/RConn1 -- SPST Switch40/LConn1
  Voltage Sensor33/RConn1 -- PS-Simulink Converter144/LConn1
  Resistor35/LConn1 -- SPST Switch39/RConn1
  EOL TWAICE Cell Model Pair 20/LConn1 -- Current Sensor55/LConn1
  PS-Simulink Converter152/LConn1 -- Voltage Sensor31/RConn1
  Simulink-PS Converter38/RConn1 -- SPST Switch36/LConn1
  SPST Switch36/RConn1 -- Resistor33/LConn1
  PS-Simulink Converter138/LConn1 -- Current Sensor51/RConn1
  Resistor36/LConn1 -- SPST Switch40/RConn1
  Resistor28/LConn1 -- SPST Switch31/RConn1
  Voltage Sensor38/RConn1 -- PS-Simulink Converter139/LConn1
  Simulink-PS Converter42/RConn1 -- SPST Switch38/LConn1
  Simulink-PS Converter43/RConn1 -- SPST Switch39/LConn1
  PS-Simulink Converter129/LConn1 -- Current Sensor58/RConn1
  Voltage Sensor29/RConn1 -- PS-Simulink Converter127/LConn1
  Simulink-PS Converter30/RConn1 -- SPST Switch28/LConn1
  Simulink-PS Converter39/RConn1 -- SPST Switch29/LConn1
  PS-Simulink Converter125/LConn1 -- Current Sensor57/RConn1
  Resistor30/LConn1 -- SPST Switch33/RConn1
  Simulink-PS Converter33/RConn1 -- SPST Switch30/LConn1
  Voltage Sensor36/RConn1 -- PS-Simulink Converter134/LConn1
  Current Sensor53/RConn1 -- PS-Simulink Converter142/LConn1
  PS-Simulink Converter147/LConn1 -- Current Sensor62/RConn1
  Current Sensor57/LConn1 -- EOL TWAICE Cell Model Pair 22/LConn1
  Current Sensor55/RConn1 -- PS-Simulink Converter155/LConn1
  BOL TWAICE Cell Model Pair 19/LConn1 -- Current Sensor54/LConn1
  PS-Simulink Converter135/LConn1 -- Voltage Sensor28/RConn1
  BOL TWAICE Cell Model Pair 13/LConn2 -- PS-Simulink Converter140/LConn1
  EOL TWAICE Cell Model Pair 24/LConn1 -- Current Sensor59/LConn1
  PS-Simulink Converter149/LConn1 -- EOL TWAICE Cell Model Pair 16/LConn2
  Resistor31/LConn1 -- SPST Switch34/RConn1
  EOL TWAICE Cell Model Pair 14/LConn1 -- Current Sensor60/LConn1
  Voltage Sensor26/RConn1 -- PS-Simulink Converter160/LConn1
  BOL TWAICE Cell Model Pair 17/LConn1 -- Current Sensor52/LConn1
  PS-Simulink Converter141/LConn1 -- Current Sensor60/RConn1
  Simulink-PS Converter37/RConn1 -- SPST Switch37/LConn1
  PS-Simulink Converter126/LConn1 -- BOL TWAICE Cell Model Pair 23/LConn2
  PS-Simulink Converter133/LConn1 -- Voltage Sensor30/RConn1
  Current Sensor62/LConn1 -- EOL TWAICE Cell Model Pair 16/LConn1
  PS-Simulink Converter145/LConn1 -- Current Sensor61/RConn1
  PS-Simulink Converter158/LConn1 -- Voltage Sensor32/RConn1
  Simulink-PS Converter36/RConn1 -- SPST Switch33/LConn1
  Simulink-PS Converter31/RConn1 -- Controlled Current Source3/RConn1
  BOL TWAICE Cell Model Pair 21/LConn1 -- Current Sensor56/LConn1
  MT42 Capacitance2/LConn1 -- Diode2/RConn1
  PS-Simulink Converter128/LConn1 -- Voltage Sensor27/RConn1
  EOL TWAICE Cell Model Pair 24/LConn2 -- PS-Simulink Converter132/LConn1
  Resistor38/LConn1 -- SPST Switch30/RConn1
  Voltage Sensor34/RConn1 -- PS-Simulink Converter159/LConn1
